simulink model "D_FB_J_classic_invdyn"  (R2020a)
settings: Solver=ode15s  StartTime=0.0  StopTime=T  MaxStep=0.01  RelTol=1e-3
values from neighbouring files (symbols this model uses):
  a1A = 0.5    [sim_D_FB_J.m]
  a1B = 0.5    [sim_D_FB_J.m]
  a2A = 0.5    [sim_D_FB_J.m]
  a2B = 0.5    [sim_D_FB_J.m]
  a3A = 0.5    [sim_D_FB_J.m]
  a3B = 0.5    [sim_D_FB_J.m]
  fv1A = 0    [sim_D_FB_J.m]
  fv1B = 0    [sim_D_FB_J.m]
  fv1p = 0    [sim_D_FB_J.m]
  fv2A = 0    [sim_D_FB_J.m]
  fv2B = 0    [sim_D_FB_J.m]
  fv2p = 0    [sim_D_FB_J.m]
  fv3A = 0    [sim_D_FB_J.m]
  fv3B = 0    [sim_D_FB_J.m]
  g0 = -9.81    [sim_D_FB_J.m]
  Ibzz = 12.1875    [sim_D_FB_J.m]
  Iczz = 33.7594    [sim_D_FB_J.m]
  Il1Azz = 0.108333    [sim_D_FB_J.m]
  Il1Bzz = 0.108333    [sim_D_FB_J.m]
  Il2Azz = 0.108333    [sim_D_FB_J.m]
  Il2Bzz = 0.108333    [sim_D_FB_J.m]
  Il3Azz = 0.108333    [sim_D_FB_J.m]
  Il3Bzz = 0.108333    [sim_D_FB_J.m]
  Kd = 5*eye(6)    [sim_D_FB_J.m]    (also in sim_second_arm_compensation.m; sim_second_arm_compensation2.m; sim_second_arm_compensation3.m = diag([5 5 5 1 1 1]))
  Kp = 5*eye(6)    [sim_D_FB_J.m]    (also in sim_second_arm_compensation.m; sim_second_arm_compensation2.m; sim_second_arm_compensation3.m = diag([5 5 5 1 1 1]))
  L = 3    [sim_D_FB_J.m]
  m_base = 100    [sim_D_FB_J.m]
  m_cavo = 45    [sim_D_FB_J.m]
  ml0 = 1000    [sim_D_FB_J.m]
  ml1A = 5    [sim_D_FB_J.m]
  ml1B = 5    [sim_D_FB_J.m]
  ml2A = 5    [sim_D_FB_J.m]
  ml2B = 5    [sim_D_FB_J.m]
  ml3A = 5    [sim_D_FB_J.m]
  ml3B = 5    [sim_D_FB_J.m]
  offA = -0.25    [sim_D_FB_J.m]
  offB = 0.25    [sim_D_FB_J.m]
  th1A_0 = -pi/2    (= -1.57079632679)    [sim_D_FB_J.m]    (also in sim_second_arm_compensation.m = 0; sim_second_arm_compensation2.m = 0; sim_second_arm_compensation3.m = -0.523598775598)
  th1B_0 = -pi/2    (= -1.57079632679)    [sim_D_FB_J.m]    (also in sim_second_arm_compensation.m = 0; sim_second_arm_compensation2.m = 0; sim_second_arm_compensation3.m = 0.523598775598)
  th2A_0 = -pi/8    (= -0.392699081699)    [sim_D_FB_J.m]    (also in sim_second_arm_compensation.m; sim_second_arm_compensation2.m; sim_second_arm_compensation3.m = 0.523598775598)
  th2B_0 = pi/8    (= 0.392699081699)    [sim_D_FB_J.m]    (also in sim_second_arm_compensation.m; sim_second_arm_compensation2.m; sim_second_arm_compensation3.m = -0.523598775598)
  th3A_0 = -pi/8    (= -0.392699081699)    [sim_D_FB_J.m]    (also in sim_second_arm_compensation.m; sim_second_arm_compensation2.m; sim_second_arm_compensation3.m = 0.523598775598)
  th3B_0 = pi/8    (= 0.392699081699)    [sim_D_FB_J.m]    (also in sim_second_arm_compensation.m; sim_second_arm_compensation2.m; sim_second_arm_compensation3.m = -0.523598775598)
undefined symbols (not defined in the file or in its folder): X, Y, Z
libraries: sm_lib x36, nesl_utility x25
(part 3 of 4)

== matlab function D_FB_J_classic_invdyn/Inverse dynamics ==
  data: y input; q input; qd input; tau output; m_cavo parameter; m_base parameter; ml1A parameter; ml2A parameter; ml3A parameter; ml1B parameter; ml2B parameter; ml3B parameter; L parameter; a1A parameter; a2A parameter; a3A parameter; a1B parameter; a2B parameter; a3B parameter; offA parameter; offB parameter; fv1p parameter; fv2p parameter; fv1A parameter; fv2A parameter; fv3A parameter; fv1B parameter; fv2B parameter; fv3B parameter; Ibzz parameter; Iczz parameter; Il1Azz parameter; Il1Bzz parameter; Il2Azz parameter; Il2Bzz parameter; Il3Azz parameter; Il3Bzz parameter; g0 parameter
function tau = fcn(y, q, qd, ...
                   m_cavo, m_base, ml1A, ml2A, ml3A, ml1B, ml2B, ml3B, ...
                   L, a1A, a2A, a3A, a1B, a2B, a3B, offA, offB, ...
                   fv1p, fv2p, fv1A, fv2A, fv3A, fv1B, fv2B, fv3B, ...
                   Ibzz, Iczz, Il1Azz, Il1Bzz, Il2Azz, Il2Bzz, Il3Azz, Il3Bzz, g0)

% Input
alfa = q(1);
beta = q(2);
th1A = q(3);
th2A = q(4);
th3A = q(5);
th1B = q(6);
th2B = q(7);
th3B = q(8);
dalfa = qd(1);
dbeta = qd(2);
dth1A = qd(3);
dth2A = qd(4);
dth3A = qd(5);
dth1B = qd(6);
dth2B = qd(7);
dth3B = qd(8);

% Matrice B
B = [ Ibzz + Iczz + Il1Azz + Il1Bzz + Il2Azz + Il2Bzz + Il3Azz + Il3Bzz + L^2*m_base + 0.2500*L^2*m_cavo + L^2*ml1A + L^2*ml1B + L^2*ml2A + L^2*ml2B + L^2*ml3A + L^2*ml3B + 0.2500*a1A^2*ml1A + a1A^2*ml2A + a1A^2*ml3A + 0.2500*a2A^2*ml2A + a2A^2*ml3A + 0.2500*a3A^2*ml3A + 0.2500*a1B^2*ml1B + a1B^2*ml2B + a1B^2*ml3B + 0.2500*a2B^2*ml2B + a2B^2*ml3B + 0.2500*a3B^2*ml3B + ml1A*offA^2 + ml2A*offA^2 + ml1B*offB^2 + ml3A*offA^2 + ml2B*offB^2 + ml3B*offB^2 + L*a1A*ml1A*cos(beta + th1A) + 2*L*a1A*ml2A*cos(beta + th1A) + 2*L*a1A*ml3A*cos(beta + th1A) + L*a1B*ml1B*cos(beta + th1B) + 2*L*a1B*ml2B*cos(beta + th1B) + 2*L*a1B*ml3B*cos(beta + th1B) + a1A*a3A*ml3A*cos(th2A + th3A) + a1B*a3B*ml3B*cos(th2B + th3B) + a2A*ml2A*offA*cos(th1A + th2A) + 2*a2A*ml3A*offA*cos(th1A + th2A) + a2B*ml2B*offB*cos(th1B + th2B) + 2*a2B*ml3B*offB*cos(th1B + th2B) + 2*L*ml1A*offA*cos(beta) + 2*L*ml2A*offA*cos(beta) + 2*L*ml1B*offB*cos(beta) + 2*L*ml3A*offA*cos(beta) + 2*L*ml2B*offB*cos(beta) + 2*L*ml3B*offB*cos(beta) + a1A*a2A*ml2A*cos(th2A) + 2*a1A*a2A*ml3A*cos(th2A) + a2A*a3A*ml3A*cos(th3A) + a1B*a2B*ml2B*cos(th2B) + 2*a1B*a2B*ml3B*cos(th2B) + a2B*a3B*ml3B*cos(th3B) + a1A*ml1A*offA*cos(th1A) + 2*a1A*ml2A*offA*cos(th1A) + 2*a1A*ml3A*offA*cos(th1A) + a1B*ml1B*offB*cos(th1B) + 2*a1B*ml2B*offB*cos(th1B) + 2*a1B*ml3B*offB*cos(th1B) + L*a2A*ml2A*cos(beta + th1A + th2A) + 2*L*a2A*ml3A*cos(beta + th1A + th2A) + L*a2B*ml2B*cos(beta + th1B + th2B) + 2*L*a2B*ml3B*cos(beta + th1B + th2B) + a3A*ml3A*offA*cos(th1A + th2A + th3A) + a3B*ml3B*offB*cos(th1B + th2B + th3B) + L*a3A*ml3A*cos(beta + th1A + th2A + th3A) + L*a3B*ml3B*cos(beta + th1B + th2B + th3B), Ibzz + Il1Azz + Il1Bzz + Il2Azz + Il2Bzz + Il3Azz + Il3Bzz + 0.2500*a1A^2*ml1A + a1A^2*ml2A + a1A^2*ml3A + 0.2500*a2A^2*ml2A + a2A^2*ml3A + 0.2500*a3A^2*ml3A + 0.2500*a1B^2*ml1B + a1B^2*ml2B + a1B^2*ml3B + 0.2500*a2B^2*ml2B + a2B^2*ml3B + 0.2500*a3B^2*ml3B + ml1A*offA^2 + ml2A*offA^2 + ml1B*offB^2 + ml3A*offA^2 + ml2B*offB^2 + ml3B*offB^2 + 0.5000*L*a1A*ml1A*cos(beta + th1A) + L*a1A*ml2A*cos(beta + th1A) + L*a1A*ml3A*cos(beta + th1A) + 0.5000*L*a1B*ml1B*cos(beta + th1B) + L*a1B*ml2B*cos(beta + th1B) + L*a1B*ml3B*cos(beta + th1B) + a1A*a3A*ml3A*cos(th2A + th3A) + a1B*a3B*ml3B*cos(th2B + th3B) + a2A*ml2A*offA*cos(th1A + th2A) + 2*a2A*ml3A*offA*cos(th1A + th2A) + a2B*ml2B*offB*cos(th1B + th2B) + 2*a2B*ml3B*offB*cos(th1B + th2B) + L*ml1A*offA*cos(beta) + L*ml2A*offA*cos(beta) + L*ml1B*offB*cos(beta) + L*ml3A*offA*cos(beta) + L*ml2B*offB*cos(beta) + L*ml3B*offB*cos(beta) + a1A*a2A*ml2A*cos(th2A) + 2*a1A*a2A*ml3A*cos(th2A) + a2A*a3A*ml3A*cos(th3A) + a1B*a2B*ml2B*cos(th2B) + 2*a1B*a2B*ml3B*cos(th2B) + a2B*a3B*ml3B*cos(th3B) + a1A*ml1A*offA*cos(th1A) + 2*a1A*ml2A*offA*cos(th1A) + 2*a1A*ml3A*offA*cos(th1A) + a1B*ml1B*offB*cos(th1B) + 2*a1B*ml2B*offB*cos(th1B) + 2*a1B*ml3B*offB*cos(th1B) + 0.5000*L*a2A*ml2A*cos(beta + th1A + th2A) + L*a2A*ml3A*cos(beta + th1A + th2A) + 0.5000*L*a2B*ml2B*cos(beta + th1B + th2B) + L*a2B*ml3B*cos(beta + th1B + th2B) + a3A*ml3A*offA*cos(th1A + th2A + th3A) + a3B*ml3B*offB*cos(th1B + th2B + th3B) + 0.5000*L*a3A*ml3A*cos(beta + th1A + th2A + th3A) + 0.5000*L*a3B*ml3B*cos(beta + th1B + th2B + th3B), Il1Azz + Il2Azz + Il3Azz + 0.2500*a1A^2*ml1A + a1A^2*ml2A + a1A^2*ml3A + 0.2500*a2A^2*ml2A + a2A^2*ml3A + 0.2500*a3A^2*ml3A + 0.5000*L*a1A*ml1A*cos(beta + th1A) + L*a1A*ml2A*cos(beta + th1A) + L*a1A*ml3A*cos(beta + th1A) + a1A*a3A*ml3A*cos(th2A + th3A) + 0.5000*a2A*ml2A*offA*cos(th1A + th2A) + a2A*ml3A*offA*cos(th1A + th2A) + a1A*a2A*ml2A*cos(th2A) + 2*a1A*a2A*ml3A*cos(th2A) + a2A*a3A*ml3A*cos(th3A) + 0.5000*a1A*ml1A*offA*cos(th1A) + a1A*ml2A*offA*cos(th1A) + a1A*ml3A*offA*cos(th1A) + 0.5000*L*a2A*ml2A*cos(beta + th1A + th2A) + L*a2A*ml3A*cos(beta + th1A + th2A) + 0.5000*a3A*ml3A*offA*cos(th1A + th2A + th3A) + 0.5000*L*a3A*ml3A*cos(beta + th1A + th2A + th3A), Il2Azz + Il3Azz + 0.2500*a2A^2*ml2A + a2A^2*ml3A + 0.2500*a3A^2*ml3A + 0.5000*a1A*a3A*ml3A*cos(th2A + th3A) + 0.5000*a2A*ml2A*offA*cos(th1A + th2A) + a2A*ml3A*offA*cos(th1A + th2A) + 0.5000*a1A*a2A*ml2A*cos(th2A) + a1A*a2A*ml3A*cos(th2A) + a2A*a3A*ml3A*cos(th3A) + 0.5000*L*a2A*ml2A*cos(beta + th1A + th2A) + L*a2A*ml3A*cos(beta + th1A + th2A) + 0.5000*a3A*ml3A*offA*cos(th1A + th2A + th3A) + 0.5000*L*a3A*ml3A*cos(beta + th1A + th2A + th3A), Il3Azz + 0.2500*a3A^2*ml3A + 0.5000*a1A*a3A*ml3A*cos(th2A + th3A) + 0.5000*a2A*a3A*ml3A*cos(th3A) + 0.5000*a3A*ml3A*offA*cos(th1A + th2A + th3A) + 0.5000*L*a3A*ml3A*cos(beta + th1A + th2A + th3A), Il1Bzz + Il2Bzz + Il3Bzz + 0.2500*a1B^2*ml1B + a1B^2*ml2B + a1B^2*ml3B + 0.2500*a2B^2*ml2B + a2B^2*ml3B + 0.2500*a3B^2*ml3B + 0.5000*L*a1B*ml1B*cos(beta + th1B) + L*a1B*ml2B*cos(beta + th1B) + L*a1B*ml3B*cos(beta + th1B) + a1B*a3B*ml3B*cos(th2B + th3B) + 0.5000*a2B*ml2B*offB*cos(th1B + th2B) + a2B*ml3B*offB*cos(th1B + th2B) + a1B*a2B*ml2B*cos(th2B) + 2*a1B*a2B*ml3B*cos(th2B) + a2B*a3B*ml3B*cos(th3B) + 0.5000*a1B*ml1B*offB*cos(th1B) + a1B*ml2B*offB*cos(th1B) + a1B*ml3B*offB*cos(th1B) + 0.5000*L*a2B*ml2B*cos(beta + th1B + th2B) + L*a2B*ml3B*cos(beta + th1B + th2B) + 0.5000*a3B*ml3B*offB*cos(th1B + th2B + th3B) + 0.5000*L*a3B*ml3B*cos(beta + th1B + th2B + th3B), Il2Bzz + Il3Bzz + 0.2500*a2B^2*ml2B + a2B^2*ml3B + 0.2500*a3B^2*ml3B + 0.5000*a1B*a3B*ml3B*cos(th2B + th3B) + 0.5000*a2B*ml2B*offB*cos(th1B + th2B) + a2B*ml3B*offB*cos(th1B + th2B) + 0.5000*a1B*a2B*ml2B*cos(th2B) + a1B*a2B*ml3B*cos(th2B) + a2B*a3B*ml3B*cos(th3B) + 0.5000*L*a2B*ml2B*cos(beta + th1B + th2B) + L*a2B*ml3B*cos(beta + th1B + th2B) + 0.5000*a3B*ml3B*offB*cos(th1B + th2B + th3B) + 0.5000*L*a3B*ml3B*cos(beta + th1B + th2B + th3B), Il3Bzz + 0.2500*a3B^2*ml3B + 0.5000*a1B*a3B*ml3B*cos(th2B + th3B) + 0.5000*a2B*a3B*ml3B*cos(th3B) + 0.5000*a3B*ml3B*offB*cos(th1B + th2B + th3B) + 0.5000*L*a3B*ml3B*cos(beta + th1B + th2B + th3B); ...
                                                                                              Ibzz + Il1Azz + Il1Bzz + Il2Azz + Il2Bzz + Il3Azz + Il3Bzz + 0.2500*a1A^2*ml1A + a1A^2*ml2A + a1A^2*ml3A + 0.2500*a2A^2*ml2A + a2A^2*ml3A + 0.2500*a3A^2*ml3A + 0.2500*a1B^2*ml1B + a1B^2*ml2B + a1B^2*ml3B + 0.2500*a2B^2*ml2B + a2B^2*ml3B + 0.2500*a3B^2*ml3B + ml1A*offA^2 + ml2A*offA^2 + ml1B*offB^2 + ml3A*offA^2 + ml2B*offB^2 + ml3B*offB^2 + 0.5000*L*a1A*ml1A*cos(beta + th1A) + L*a1A*ml2A*cos(beta + th1A) + L*a1A*ml3A*cos(beta + th1A) + 0.5000*L*a1B*ml1B*cos(beta + th1B) + L*a1B*ml2B*cos(beta + th1B) + L*a1B*ml3B*cos(beta + th1B) + a1A*a3A*ml3A*cos(th2A + th3A) + a1B*a3B*ml3B*cos(th2B + th3B) + a2A*ml2A*offA*cos(th1A + th2A) + 2*a2A*ml3A*offA*cos(th1A + th2A) + a2B*ml2B*offB*cos(th1B + th2B) + 2*a2B*ml3B*offB*cos(th1B + th2B) + L*ml1A*offA*cos(beta) + L*ml2A*offA*cos(beta) + L*ml1B*offB*cos(beta) + L*ml3A*offA*cos(beta) + L*ml2B*offB*cos(beta) + L*ml3B*offB*cos(beta) + a1A*a2A*ml2A*cos(th2A) + 2*a1A*a2A*ml3A*cos(th2A) + a2A*a3A*ml3A*cos(th3A) + a1B*a2B*ml2B*cos(th2B) + 2*a1B*a2B*ml3B*cos(th2B) + a2B*a3B*ml3B*cos(th3B) + a1A*ml1A*offA*cos(th1A) + 2*a1A*ml2A*offA*cos(th1A) + 2*a1A*ml3A*offA*cos(th1A) + a1B*ml1B*offB*cos(th1B) + 2*a1B*ml2B*offB*cos(th1B) + 2*a1B*ml3B*offB*cos(th1B) + 0.5000*L*a2A*ml2A*cos(beta + th1A + th2A) + L*a2A*ml3A*cos(beta + th1A + th2A) + 0.5000*L*a2B*ml2B*cos(beta + th1B + th2B) + L*a2B*ml3B*cos(beta + th1B + th2B) + a3A*ml3A*offA*cos(th1A + th2A + th3A) + a3B*ml3B*offB*cos(th1B + th2B + th3B) + 0.5000*L*a3A*ml3A*cos(beta + th1A + th2A + th3A) + 0.5000*L*a3B*ml3B*cos(beta + th1B + th2B + th3B),                                                                                                                                                                                                                                                                                                                                                                                                                                                                                                                                                                                                                           Ibzz + Il1Azz + Il1Bzz + Il2Azz + Il2Bzz + Il3Azz + Il3Bzz + 0.2500*a1A^2*ml1A + a1A^2*ml2A + a1A^2*ml3A + 0.2500*a2A^2*ml2A + a2A^2*ml3A + 0.2500*a3A^2*ml3A + 0.2500*a1B^2*ml1B + a1B^2*ml2B + a1B^2*ml3B + 0.2500*a2B^2*ml2B + a2B^2*ml3B + 0.2500*a3B^2*ml3B + ml1A*offA^2 + ml2A*offA^2 + ml1B*offB^2 + ml3A*offA^2 + ml2B*offB^2 + ml3B*offB^2 + a1A*a3A*ml3A*cos(th2A + th3A) + a1B*a3B*ml3B*cos(th2B + th3B) + a2A*ml2A*offA*cos(th1A + th2A) + 2*a2A*ml3A*offA*cos(th1A + th2A) + a2B*ml2B*offB*cos(th1B + th2B) + 2*a2B*ml3B*offB*cos(th1B + th2B) + a1A*a2A*ml2A*cos(th2A) + 2*a1A*a2A*ml3A*cos(th2A) + a2A*a3A*ml3A*cos(th3A) + a1B*a2B*ml2B*cos(th2B) + 2*a1B*a2B*ml3B*cos(th2B) + a2B*a3B*ml3B*cos(th3B) + a1A*ml1A*offA*cos(th1A) + 2*a1A*ml2A*offA*cos(th1A) + 2*a1A*ml3A*offA*cos(th1A) + a1B*ml1B*offB*cos(th1B) + 2*a1B*ml2B*offB*cos(th1B) + 2*a1B*ml3B*offB*cos(th1B) + a3A*ml3A*offA*cos(th1A + th2A + th3A) + a3B*ml3B*offB*cos(th1B + th2B + th3B),                                                                                                                                                                                                                                      Il1Azz + Il2Azz + Il3Azz + 0.2500*a1A^2*ml1A + a1A^2*ml2A + a1A^2*ml3A + 0.2500*a2A^2*ml2A + a2A^2*ml3A + 0.2500*a3A^2*ml3A + a1A*a3A*ml3A*cos(th2A + th3A) + 0.5000*a2A*ml2A*offA*cos(th1A + th2A) + a2A*ml3A*offA*cos(th1A + th2A) + a1A*a2A*ml2A*cos(th2A) + 2*a1A*a2A*ml3A*cos(th2A) + a2A*a3A*ml3A*cos(th3A) + 0.5000*a1A*ml1A*offA*cos(th1A) + a1A*ml2A*offA*cos(th1A) + a1A*ml3A*offA*cos(th1A) + 0.5000*a3A*ml3A*offA*cos(th1A + th2A + th3A),                                                                                                                                     Il2Azz + Il3Azz + 0.2500*a2A^2*ml2A + a2A^2*ml3A + 0.2500*a3A^2*ml3A + 0.5000*a1A*a3A*ml3A*cos(th2A + th3A) + 0.5000*a2A*ml2A*offA*cos(th1A + th2A) + a2A*ml3A*offA*cos(th1A + th2A) + 0.5000*a1A*a2A*ml2A*cos(th2A) + a1A*a2A*ml3A*cos(th2A) + a2A*a3A*ml3A*cos(th3A) + 0.5000*a3A*ml3A*offA*cos(th1A + th2A + th3A),                                                    Il3Azz + 0.2500*a3A^2*ml3A + 0.5000*a1A*a3A*ml3A*cos(th2A + th3A) + 0.5000*a2A*a3A*ml3A*cos(th3A) + 0.5000*a3A*ml3A*offA*cos(th1A + th2A + th3A),                                                                                                                                                                                                                                      Il1Bzz + Il2Bzz + Il3Bzz + 0.2500*a1B^2*ml1B + a1B^2*ml2B + a1B^2*ml3B + 0.2500*a2B^2*ml2B + a2B^2*ml3B + 0.2500*a3B^2*ml3B + a1B*a3B*ml3B*cos(th2B + th3B) + 0.5000*a2B*ml2B*offB*cos(th1B + th2B) + a2B*ml3B*offB*cos(th1B + th2B) + a1B*a2B*ml2B*cos(th2B) + 2*a1B*a2B*ml3B*cos(th2B) + a2B*a3B*ml3B*cos(th3B) + 0.5000*a1B*ml1B*offB*cos(th1B) + a1B*ml2B*offB*cos(th1B) + a1B*ml3B*offB*cos(th1B) + 0.5000*a3B*ml3B*offB*cos(th1B + th2B + th3B),                                                                                                                                     Il2Bzz + Il3Bzz + 0.2500*a2B^2*ml2B + a2B^2*ml3B + 0.2500*a3B^2*ml3B + 0.5000*a1B*a3B*ml3B*cos(th2B + th3B) + 0.5000*a2B*ml2B*offB*cos(th1B + th2B) + a2B*ml3B*offB*cos(th1B + th2B) + 0.5000*a1B*a2B*ml2B*cos(th2B) + a1B*a2B*ml3B*cos(th2B) + a2B*a3B*ml3B*cos(th3B) + 0.5000*a3B*ml3B*offB*cos(th1B + th2B + th3B),                                                    Il3Bzz + 0.2500*a3B^2*ml3B + 0.5000*a1B*a3B*ml3B*cos(th2B + th3B) + 0.5000*a2B*a3B*ml3B*cos(th3B) + 0.5000*a3B*ml3B*offB*cos(th1B + th2B + th3B); ...
                                                                                                                                                                                                                                                                                                                                                                                                                                                                                                                                                                                                                                                                                                                                                                                                                                                                                                                                                                                                        Il1Azz + Il2Azz + Il3Azz + 0.2500*a1A^2*ml1A + a1A^2*ml2A + a1A^2*ml3A + 0.2500*a2A^2*ml2A + a2A^2*ml3A + 0.2500*a3A^2*ml3A + 0.5000*L*a1A*ml1A*cos(beta + th1A) + L*a1A*ml2A*cos(beta + th1A) + L*a1A*ml3A*cos(beta + th1A) + a1A*a3A*ml3A*cos(th2A + th3A) + 0.5000*a2A*ml2A*offA*cos(th1A + th2A) + a2A*ml3A*offA*cos(th1A + th2A) + a1A*a2A*ml2A*cos(th2A) + 2*a1A*a2A*ml3A*cos(th2A) + a2A*a3A*ml3A*cos(th3A) + 0.5000*a1A*ml1A*offA*cos(th1A) + a1A*ml2A*offA*cos(th1A) + a1A*ml3A*offA*cos(th1A) + 0.5000*L*a2A*ml2A*cos(beta + th1A + th2A) + L*a2A*ml3A*cos(beta + th1A + th2A) + 0.5000*a3A*ml3A*offA*cos(th1A + th2A + th3A) + 0.5000*L*a3A*ml3A*cos(beta + th1A + th2A + th3A),                                                                                                                                                                                                                                                                                                                                                                                                                                                                                                                                                                                                                                                                                                                                                                                                                                                                                                                                                                                                                                                                                                                                                Il1Azz + Il2Azz + Il3Azz + 0.2500*a1A^2*ml1A + a1A^2*ml2A + a1A^2*ml3A + 0.2500*a2A^2*ml2A + a2A^2*ml3A + 0.2500*a3A^2*ml3A + a1A*a3A*ml3A*cos(th2A + th3A) + 0.5000*a2A*ml2A*offA*cos(th1A + th2A) + a2A*ml3A*offA*cos(th1A + th2A) + a1A*a2A*ml2A*cos(th2A) + 2*a1A*a2A*ml3A*cos(th2A) + a2A*a3A*ml3A*cos(th3A) + 0.5000*a1A*ml1A*offA*cos(th1A) + a1A*ml2A*offA*cos(th1A) + a1A*ml3A*offA*cos(th1A) + 0.5000*a3A*ml3A*offA*cos(th1A + th2A + th3A),                                                                                                                                                                                                                                                                                                                                                                                                                                                   Il1Azz + Il2Azz + Il3Azz + 0.2500*a1A^2*ml1A + a1A^2*ml2A + a1A^2*ml3A + 0.2500*a2A^2*ml2A + a2A^2*ml3A + 0.2500*a3A^2*ml3A + a1A*a3A*ml3A*cos(th2A + th3A) + a1A*a2A*ml2A*cos(th2A) + 2*a1A*a2A*ml3A*cos(th2A) + a2A*a3A*ml3A*cos(th3A),                                                                                                                                                                                                                                                             Il2Azz + Il3Azz + 0.2500*a2A^2*ml2A + a2A^2*ml3A + 0.2500*a3A^2*ml3A + 0.5000*a1A*a3A*ml3A*cos(th2A + th3A) + 0.5000*a1A*a2A*ml2A*cos(th2A) + a1A*a2A*ml3A*cos(th2A) + a2A*a3A*ml3A*cos(th3A),                                                                                                   Il3Azz + 0.2500*a3A^2*ml3A + 0.5000*a1A*a3A*ml3A*cos(th2A + th3A) + 0.5000*a2A*a3A*ml3A*cos(th3A),                                                                                                                                                                                                                                                                                                                                                                                                                                                                                                                                                                                                                                                                                          0,                                                                                                                                                                                                                                                                                                                                                                                                                                                         0,                                                                                                                                                                                                   0; ...
                                                                                                                                                                                                                                                                                                                                                                                                                                                                                                                                                                                                                                                                                                                                                                                                                                                                                                                                                                                                                                                                                                                                                                                                                                         Il2Azz + Il3Azz + 0.2500*a2A^2*ml2A + a2A^2*ml3A + 0.2500*a3A^2*ml3A + 0.5000*a1A*a3A*ml3A*cos(th2A + th3A) + 0.5000*a2A*ml2A*offA*cos(th1A + th2A) + a2A*ml3A*offA*cos(th1A + th2A) + 0.5000*a1A*a2A*ml2A*cos(th2A) + a1A*a2A*ml3A*cos(th2A) + a2A*a3A*ml3A*cos(th3A) + 0.5000*L*a2A*ml2A*cos(beta + th1A + th2A) + L*a2A*ml3A*cos(beta + th1A + th2A) + 0.5000*a3A*ml3A*offA*cos(th1A + th2A + th3A) + 0.5000*L*a3A*ml3A*cos(beta + th1A + th2A + th3A),                                                                                                                                                                                                                                                                                                                                                                                                                                                                                                                                                                                                                                                                                                                                                                                                                                                                                                                                                                                                                                                                                                                                                                                                                                                                                Il2Azz + Il3Azz + 0.2500*a2A^2*ml2A + a2A^2*ml3A + 0.2500*a3A^2*ml3A + 0.5000*a1A*a3A*ml3A*cos(th2A + th3A) + 0.5000*a2A*ml2A*offA*cos(th1A + th2A) + a2A*ml3A*offA*cos(th1A + th2A) + 0.5000*a1A*a2A*ml2A*cos(th2A) + a1A*a2A*ml3A*cos(th2A) + a2A*a3A*ml3A*cos(th3A) + 0.5000*a3A*ml3A*offA*cos(th1A + th2A + th3A),                                                                                                                                                                                                                                                                                                                                                                                                                                                                                              Il2Azz + Il3Azz + 0.2500*a2A^2*ml2A + a2A^2*ml3A + 0.2500*a3A^2*ml3A + 0.5000*a1A*a3A*ml3A*cos(th2A + th3A) + 0.5000*a1A*a2A*ml2A*cos(th2A) + a1A*a2A*ml3A*cos(th2A) + a2A*a3A*ml3A*cos(th3A),                                                                                                                                                                                                                                                                                                                                                             Il2Azz + Il3Azz + 0.2500*a2A^2*ml2A + a2A^2*ml3A + 0.2500*a3A^2*ml3A + a2A*a3A*ml3A*cos(th3A),                                                                                                                                          0.2500*ml3A*a3A^2 + 0.5000*a2A*ml3A*cos(th3A)*a3A + Il3Azz,                                                                                                                                                                                                                                                                                                                                                                                                                                                                                                                                                                                                                                                                                          0,                                                                                                                                                                                                                                                                                                                                                                                                                                                         0,                                                                                                                                                                                                   0; ...
                                                                                                                                                                                                                                                                                                                                                                                                                                                                                                                                                                                                                                                                                                                                                                                                                                                                                                                                                                                                                                                                                                                                                                                                                                                                                                                                                                                                                                                                                               Il3Azz + 0.2500*a3A^2*ml3A + 0.5000*a1A*a3A*ml3A*cos(th2A + th3A) + 0.5000*a2A*a3A*ml3A*cos(th3A) + 0.5000*a3A*ml3A*offA*cos(th1A + th2A + th3A) + 0.5000*L*a3A*ml3A*cos(beta + th1A + th2A + th3A),                                                                                                                                                                                                                                                                                                                                                                                                                                                                                                                                                                                                                                                                                                                                                                                                                                                                                                                                                                                                                                                                                                                                                                                                                                                                                                                                                                                                                                                     Il3Azz + 0.2500*a3A^2*ml3A + 0.5000*a1A*a3A*ml3A*cos(th2A + th3A) + 0.5000*a2A*a3A*ml3A*cos(th3A) + 0.5000*a3A*ml3A*offA*cos(th1A + th2A + th3A),                                                                                                                                                                                                                                                                                                                                                                                                                                                                                                                                                                                          Il3Azz + 0.2500*a3A^2*ml3A + 0.5000*a1A*a3A*ml3A*cos(th2A + th3A) + 0.5000*a2A*a3A*ml3A*cos(th3A),                                                                                                                                                                                                                                                                                                                                                                                                0.2500*ml3A*a3A^2 + 0.5000*a2A*ml3A*cos(th3A)*a3A + Il3Azz,                                                                                                                                                                          0.2500*ml3A*a3A^2 + Il3Azz,                                                                                                                                                                                                                                                                                                                                                                                                                                                                                                                                                                                                                                                                                          0,                                                                                                                                                                                                                                                                                                                                                                                                                                                         0,                                                                                                                                                                                                   0; ...
                                                                                                                                                                                                                                                                                                                                                                                                                                                                                                                                                                                                                                                                                                                                                                                                                                                                                                                                                                                                        Il1Bzz + Il2Bzz + Il3Bzz + 0.2500*a1B^2*ml1B + a1B^2*ml2B + a1B^2*ml3B + 0.2500*a2B^2*ml2B + a2B^2*ml3B + 0.2500*a3B^2*ml3B + 0.5000*L*a1B*ml1B*cos(beta + th1B) + L*a1B*ml2B*cos(beta + th1B) + L*a1B*ml3B*cos(beta + th1B) + a1B*a3B*ml3B*cos(th2B + th3B) + 0.5000*a2B*ml2B*offB*cos(th1B + th2B) + a2B*ml3B*offB*cos(th1B + th2B) + a1B*a2B*ml2B*cos(th2B) + 2*a1B*a2B*ml3B*cos(th2B) + a2B*a3B*ml3B*cos(th3B) + 0.5000*a1B*ml1B*offB*cos(th1B) + a1B*ml2B*offB*cos(th1B) + a1B*ml3B*offB*cos(th1B) + 0.5000*L*a2B*ml2B*cos(beta + th1B + th2B) + L*a2B*ml3B*cos(beta + th1B + th2B) + 0.5000*a3B*ml3B*offB*cos(th1B + th2B + th3B) + 0.5000*L*a3B*ml3B*cos(beta + th1B + th2B + th3B),                                                                                                                                                                                                                                                                                                                                                                                                                                                                                                                                                                                                                                                                                                                                                                                                                                                                                                                                                                                                                                                                                                                                                Il1Bzz + Il2Bzz + Il3Bzz + 0.2500*a1B^2*ml1B + a1B^2*ml2B + a1B^2*ml3B + 0.2500*a2B^2*ml2B + a2B^2*ml3B + 0.2500*a3B^2*ml3B + a1B*a3B*ml3B*cos(th2B + th3B) + 0.5000*a2B*ml2B*offB*cos(th1B + th2B) + a2B*ml3B*offB*cos(th1B + th2B) + a1B*a2B*ml2B*cos(th2B) + 2*a1B*a2B*ml3B*cos(th2B) + a2B*a3B*ml3B*cos(th3B) + 0.5000*a1B*ml1B*offB*cos(th1B) + a1B*ml2B*offB*cos(th1B) + a1B*ml3B*offB*cos(th1B) + 0.5000*a3B*ml3B*offB*cos(th1B + th2B + th3B),                                                                                                                                                                                                                                                                                                                                                                                                                                                                                                                                                                                                                                                                                          0,                                                                                                                                                                                                                                                                                                                                                                                                                                                         0,                                                                                                                                                                                                   0,                                                                                                                                                                                                                                                                                                                                                                                                                                                   Il1Bzz + Il2Bzz + Il3Bzz + 0.2500*a1B^2*ml1B + a1B^2*ml2B + a1B^2*ml3B + 0.2500*a2B^2*ml2B + a2B^2*ml3B + 0.2500*a3B^2*ml3B + a1B*a3B*ml3B*cos(th2B + th3B) + a1B*a2B*ml2B*cos(th2B) + 2*a1B*a2B*ml3B*cos(th2B) + a2B*a3B*ml3B*cos(th3B),                                                                                                                                                                                                                                                             Il2Bzz + Il3Bzz + 0.2500*a2B^2*ml2B + a2B^2*ml3B + 0.2500*a3B^2*ml3B + 0.5000*a1B*a3B*ml3B*cos(th2B + th3B) + 0.5000*a1B*a2B*ml2B*cos(th2B) + a1B*a2B*ml3B*cos(th2B) + a2B*a3B*ml3B*cos(th3B),                                                                                                   Il3Bzz + 0.2500*a3B^2*ml3B + 0.5000*a1B*a3B*ml3B*cos(th2B + th3B) + 0.5000*a2B*a3B*ml3B*cos(th3B); ...
                                                                                                                                                                                                                                                                                                                                                                                                                                                                                                                                                                                                                                                                                                                                                                                                                                                                                                                                                                                                                                                                                                                                                                                                                                         Il2Bzz + Il3Bzz + 0.2500*a2B^2*ml2B + a2B^2*ml3B + 0.2500*a3B^2*ml3B + 0.5000*a1B*a3B*ml3B*cos(th2B + th3B) + 0.5000*a2B*ml2B*offB*cos(th1B + th2B) + a2B*ml3B*offB*cos(th1B + th2B) + 0.5000*a1B*a2B*ml2B*cos(th2B) + a1B*a2B*ml3B*cos(th2B) + a2B*a3B*ml3B*cos(th3B) + 0.5000*L*a2B*ml2B*cos(beta + th1B + th2B) + L*a2B*ml3B*cos(beta + th1B + th2B) + 0.5000*a3B*ml3B*offB*cos(th1B + th2B + th3B) + 0.5000*L*a3B*ml3B*cos(beta + th1B + th2B + th3B),                                                                                                                                                                                                                                                                                                                                                                                                                                                                                                                                                                                                                                                                                                                                                                                                                                                                                                                                                                                                                                                                                                                                                                                                                                                                                Il2Bzz + Il3Bzz + 0.2500*a2B^2*ml2B + a2B^2*ml3B + 0.2500*a3B^2*ml3B + 0.5000*a1B*a3B*ml3B*cos(th2B + th3B) + 0.5000*a2B*ml2B*offB*cos(th1B + th2B) + a2B*ml3B*offB*cos(th1B + th2B) + 0.5000*a1B*a2B*ml2B*cos(th2B) + a1B*a2B*ml3B*cos(th2B) + a2B*a3B*ml3B*cos(th3B) + 0.5000*a3B*ml3B*offB*cos(th1B + th2B + th3B),                                                                                                                                                                                                                                                                                                                                                                                                                                                                                                                                                                                                                                                                                          0,                                                                                                                                                                                                                                                                                                                                                                                                                                                         0,                                                                                                                                                                                                   0,                                                                                                                                                                                                                                                                                                                                                                                                                                                                                              Il2Bzz + Il3Bzz + 0.2500*a2B^2*ml2B + a2B^2*ml3B + 0.2500*a3B^2*ml3B + 0.5000*a1B*a3B*ml3B*cos(th2B + th3B) + 0.5000*a1B*a2B*ml2B*cos(th2B) + a1B*a2B*ml3B*cos(th2B) + a2B*a3B*ml3B*cos(th3B),                                                                                                                                                                                                                                                                                                                                                             Il2Bzz + Il3Bzz + 0.2500*a2B^2*ml2B + a2B^2*ml3B + 0.2500*a3B^2*ml3B + a2B*a3B*ml3B*cos(th3B),                                                                                                                                          0.2500*ml3B*a3B^2 + 0.5000*a2B*ml3B*cos(th3B)*a3B + Il3Bzz; ...
                                                                                                                                                                                                                                                                                                                                                                                                                                                                                                                                                                                                                                                                                                                                                                                                                                                                                                                                                                                                                                                                                                                                                                                                                                                                                                                                                                                                                                                                                               Il3Bzz + 0.2500*a3B^2*ml3B + 0.5000*a1B*a3B*ml3B*cos(th2B + th3B) + 0.5000*a2B*a3B*ml3B*cos(th3B) + 0.5000*a3B*ml3B*offB*cos(th1B + th2B + th3B) + 0.5000*L*a3B*ml3B*cos(beta + th1B + th2B + th3B),                                                                                                                                                                                                                                                                                                                                                                                                                                                                                                                                                                                                                                                                                                                                                                                                                                                                                                                                                                                                                                                                                                                                                                                                                                                                                                                                                                                                                                                     Il3Bzz + 0.2500*a3B^2*ml3B + 0.5000*a1B*a3B*ml3B*cos(th2B + th3B) + 0.5000*a2B*a3B*ml3B*cos(th3B) + 0.5000*a3B*ml3B*offB*cos(th1B + th2B + th3B),                                                                                                                                                                                                                                                                                                                                                                                                                                                                                                                                                                                                                                                                                          0,                                                                                                                                                                                                                                                                                                                                                                                                                                                         0,                                                                                                                                                                                                   0,                                                                                                                                                                                                                                                                                                                                                                                                                                                                                                                                                                                          Il3Bzz + 0.2500*a3B^2*ml3B + 0.5000*a1B*a3B*ml3B*cos(th2B + th3B) + 0.5000*a2B*a3B*ml3B*cos(th3B),                                                                                                                                                                                                                                                                                                                                                                                                0.2500*ml3B*a3B^2 + 0.5000*a2B*ml3B*cos(th3B)*a3B + Il3Bzz,                                                                                                                                                                          0.2500*ml3B*a3B^2 + Il3Bzz];
 
% Matrice C
C = [ - 0.5000*a3A*dth1A*ml3A*offA*sin(th1A + th2A + th3A) - 0.5000*a3A*dth2A*ml3A*offA*sin(th1A + th2A + th3A) - 0.5000*a3A*dth3A*ml3A*offA*sin(th1A + th2A + th3A) - 0.5000*a3B*dth1B*ml3B*offB*sin(th1B + th2B + th3B) - 0.5000*a3B*dth2B*ml3B*offB*sin(th1B + th2B + th3B) - 0.5000*a3B*dth3B*ml3B*offB*sin(th1B + th2B + th3B) - 0.5000*L*a3A*dbeta*ml3A*sin(beta + th1A + th2A + th3A) - 0.5000*L*a3B*dbeta*ml3B*sin(beta + th1B + th2B + th3B) - 0.5000*L*a3A*dth1A*ml3A*sin(beta + th1A + th2A + th3A) - 0.5000*L*a3A*dth2A*ml3A*sin(beta + th1A + th2A + th3A) - 0.5000*L*a3A*dth3A*ml3A*sin(beta + th1A + th2A + th3A) - 0.5000*L*a3B*dth1B*ml3B*sin(beta + th1B + th2B + th3B) - 0.5000*L*a3B*dth2B*ml3B*sin(beta + th1B + th2B + th3B) - 0.5000*L*a3B*dth3B*ml3B*sin(beta + th1B + th2B + th3B) - 0.5000*L*a1A*dbeta*ml1A*sin(beta + th1A) - L*a1A*dbeta*ml2A*sin(beta + th1A) - L*a1A*dbeta*ml3A*sin(beta + th1A) - 0.5000*L*a1B*dbeta*ml1B*sin(beta + th1B) - L*a1B*dbeta*ml2B*sin(beta + th1B) - L*a1B*dbeta*ml3B*sin(beta + th1B) - 0.5000*L*a1A*dth1A*ml1A*sin(beta + th1A) - L*a1A*dth1A*ml2A*sin(beta + th1A) - L*a1A*dth1A*ml3A*sin(beta + th1A) - 0.5000*L*a1B*dth1B*ml1B*sin(beta + th1B) - L*a1B*dth1B*ml2B*sin(beta + th1B) - L*a1B*dth1B*ml3B*sin(beta + th1B) - 0.5000*a1A*a3A*dth2A*ml3A*sin(th2A + th3A) - 0.5000*a1A*a3A*dth3A*ml3A*sin(th2A + th3A) - 0.5000*a1B*a3B*dth2B*ml3B*sin(th2B + th3B) - 0.5000*a1B*a3B*dth3B*ml3B*sin(th2B + th3B) - 0.5000*a2A*dth1A*ml2A*offA*sin(th1A + th2A) - a2A*dth1A*ml3A*offA*sin(th1A + th2A) - 0.5000*a2A*dth2A*ml2A*offA*sin(th1A + th2A) - a2A*dth2A*ml3A*offA*sin(th1A + th2A) - 0.5000*a2B*dth1B*ml2B*offB*sin(th1B + th2B) - a2B*dth1B*ml3B*offB*sin(th1B + th2B) - 0.5000*a2B*dth2B*ml2B*offB*sin(th1B + th2B) - a2B*dth2B*ml3B*offB*sin(th1B + th2B) - L*dbeta*ml1A*offA*sin(beta) - L*dbeta*ml2A*offA*sin(beta) - L*dbeta*ml1B*offB*sin(beta) - L*dbeta*ml3A*offA*sin(beta) - L*dbeta*ml2B*offB*sin(beta) - L*dbeta*ml3B*offB*sin(beta) - 0.5000*a1A*a2A*dth2A*ml2A*sin(th2A) - a1A*a2A*dth2A*ml3A*sin(th2A) - 0.5000*a2A*a3A*dth3A*ml3A*sin(th3A) - 0.5000*a1B*a2B*dth2B*ml2B*sin(th2B) - a1B*a2B*dth2B*ml3B*sin(th2B) - 0.5000*a2B*a3B*dth3B*ml3B*sin(th3B) - 0.5000*a1A*dth1A*ml1A*offA*sin(th1A) - a1A*dth1A*ml2A*offA*sin(th1A) - a1A*dth1A*ml3A*offA*sin(th1A) - 0.5000*a1B*dth1B*ml1B*offB*sin(th1B) - a1B*dth1B*ml2B*offB*sin(th1B) - a1B*dth1B*ml3B*offB*sin(th1B) - 0.5000*L*a2A*dbeta*ml2A*sin(beta + th1A + th2A) - L*a2A*dbeta*ml3A*sin(beta + th1A + th2A) - 0.5000*L*a2B*dbeta*ml2B*sin(beta + th1B + th2B) - L*a2B*dbeta*ml3B*sin(beta + th1B + th2B) - 0.5000*L*a2A*dth1A*ml2A*sin(beta + th1A + th2A) - L*a2A*dth1A*ml3A*sin(beta + th1A + th2A) - 0.5000*L*a2A*dth2A*ml2A*sin(beta + th1A + th2A) - L*a2A*dth2A*ml3A*sin(beta + th1A + th2A) - 0.5000*L*a2B*dth1B*ml2B*sin(beta + th1B + th2B) - L*a2B*dth1B*ml3B*sin(beta + th1B + th2B) - 0.5000*L*a2B*dth2B*ml2B*sin(beta + th1B + th2B) - L*a2B*dth2B*ml3B*sin(beta + th1B + th2B), - 0.5000*a3A*dth1A*ml3A*offA*sin(th1A + th2A + th3A) - 0.5000*a3A*dth2A*ml3A*offA*sin(th1A + th2A + th3A) - 0.5000*a3A*dth3A*ml3A*offA*sin(th1A + th2A + th3A) - 0.5000*a3B*dth1B*ml3B*offB*sin(th1B + th2B + th3B) - 0.5000*a3B*dth2B*ml3B*offB*sin(th1B + th2B + th3B) - 0.5000*a3B*dth3B*ml3B*offB*sin(th1B + th2B + th3B) - 0.5000*L*a3A*dalfa*ml3A*sin(beta + th1A + th2A + th3A) - 0.5000*L*a3B*dalfa*ml3B*sin(beta + th1B + th2B + th3B) - 0.5000*L*a3A*dbeta*ml3A*sin(beta + th1A + th2A + th3A) - 0.5000*L*a3B*dbeta*ml3B*sin(beta + th1B + th2B + th3B) - 0.5000*L*a3A*dth1A*ml3A*sin(beta + th1A + th2A + th3A) - 0.5000*L*a3A*dth2A*ml3A*sin(beta + th1A + th2A + th3A) - 0.5000*L*a3A*dth3A*ml3A*sin(beta + th1A + th2A + th3A) - 0.5000*L*a3B*dth1B*ml3B*sin(beta + th1B + th2B + th3B) - 0.5000*L*a3B*dth2B*ml3B*sin(beta + th1B + th2B + th3B) - 0.5000*L*a3B*dth3B*ml3B*sin(beta + th1B + th2B + th3B) - 0.5000*L*a1A*dalfa*ml1A*sin(beta + th1A) - L*a1A*dalfa*ml2A*sin(beta + th1A) - L*a1A*dalfa*ml3A*sin(beta + th1A) - 0.5000*L*a1B*dalfa*ml1B*sin(beta + th1B) - L*a1B*dalfa*ml2B*sin(beta + th1B) - L*a1B*dalfa*ml3B*sin(beta + th1B) - 0.5000*L*a1A*dbeta*ml1A*sin(beta + th1A) - L*a1A*dbeta*ml2A*sin(beta + th1A) - L*a1A*dbeta*ml3A*sin(beta + th1A) - 0.5000*L*a1B*dbeta*ml1B*sin(beta + th1B) - L*a1B*dbeta*ml2B*sin(beta + th1B) - L*a1B*dbeta*ml3B*sin(beta + th1B) - 0.5000*L*a1A*dth1A*ml1A*sin(beta + th1A) - L*a1A*dth1A*ml2A*sin(beta + th1A) - L*a1A*dth1A*ml3A*sin(beta + th1A) - 0.5000*L*a1B*dth1B*ml1B*sin(beta + th1B) - L*a1B*dth1B*ml2B*sin(beta + th1B) - L*a1B*dth1B*ml3B*sin(beta + th1B) - 0.5000*a1A*a3A*dth2A*ml3A*sin(th2A + th3A) - 0.5000*a1A*a3A*dth3A*ml3A*sin(th2A + th3A) - 0.5000*a1B*a3B*dth2B*ml3B*sin(th2B + th3B) - 0.5000*a1B*a3B*dth3B*ml3B*sin(th2B + th3B) - 0.5000*a2A*dth1A*ml2A*offA*sin(th1A + th2A) - a2A*dth1A*ml3A*offA*sin(th1A + th2A) - 0.5000*a2A*dth2A*ml2A*offA*sin(th1A + th2A) - a2A*dth2A*ml3A*offA*sin(th1A + th2A) - 0.5000*a2B*dth1B*ml2B*offB*sin(th1B + th2B) - a2B*dth1B*ml3B*offB*sin(th1B + th2B) - 0.5000*a2B*dth2B*ml2B*offB*sin(th1B + th2B) - a2B*dth2B*ml3B*offB*sin(th1B + th2B) - L*dalfa*ml1A*offA*sin(beta) - L*dalfa*ml2A*offA*sin(beta) - L*dalfa*ml1B*offB*sin(beta) - L*dalfa*ml3A*offA*sin(beta) - L*dalfa*ml2B*offB*sin(beta) - L*dalfa*ml3B*offB*sin(beta) - L*dbeta*ml1A*offA*sin(beta) - L*dbeta*ml2A*offA*sin(beta) - L*dbeta*ml1B*offB*sin(beta) - L*dbeta*ml3A*offA*sin(beta) - L*dbeta*ml2B*offB*sin(beta) - L*dbeta*ml3B*offB*sin(beta) - 0.5000*a1A*a2A*dth2A*ml2A*sin(th2A) - a1A*a2A*dth2A*ml3A*sin(th2A) - 0.5000*a2A*a3A*dth3A*ml3A*sin(th3A) - 0.5000*a1B*a2B*dth2B*ml2B*sin(th2B) - a1B*a2B*dth2B*ml3B*sin(th2B) - 0.5000*a2B*a3B*dth3B*ml3B*sin(th3B) - 0.5000*a1A*dth1A*ml1A*offA*sin(th1A) - a1A*dth1A*ml2A*offA*sin(th1A) - a1A*dth1A*ml3A*offA*sin(th1A) - 0.5000*a1B*dth1B*ml1B*offB*sin(th1B) - a1B*dth1B*ml2B*offB*sin(th1B) - a1B*dth1B*ml3B*offB*sin(th1B) - 0.5000*L*a2A*dalfa*ml2A*sin(beta + th1A + th2A) - L*a2A*dalfa*ml3A*sin(beta + th1A + th2A) - 0.5000*L*a2B*dalfa*ml2B*sin(beta + th1B + th2B) - L*a2B*dalfa*ml3B*sin(beta + th1B + th2B) - 0.5000*L*a2A*dbeta*ml2A*sin(beta + th1A + th2A) - L*a2A*dbeta*ml3A*sin(beta + th1A + th2A) - 0.5000*L*a2B*dbeta*ml2B*sin(beta + th1B + th2B) - L*a2B*dbeta*ml3B*sin(beta + th1B + th2B) - 0.5000*L*a2A*dth1A*ml2A*sin(beta + th1A + th2A) - L*a2A*dth1A*ml3A*sin(beta + th1A + th2A) - 0.5000*L*a2A*dth2A*ml2A*sin(beta + th1A + th2A) - L*a2A*dth2A*ml3A*sin(beta + th1A + th2A) - 0.5000*L*a2B*dth1B*ml2B*sin(beta + th1B + th2B) - L*a2B*dth1B*ml3B*sin(beta + th1B + th2B) - 0.5000*L*a2B*dth2B*ml2B*sin(beta + th1B + th2B) - L*a2B*dth2B*ml3B*sin(beta + th1B + th2B), - 0.5000*a3A*dalfa*ml3A*offA*sin(th1A + th2A + th3A) - 0.5000*a3A*dbeta*ml3A*offA*sin(th1A + th2A + th3A) - 0.5000*a3A*dth1A*ml3A*offA*sin(th1A + th2A + th3A) - 0.5000*a3A*dth2A*ml3A*offA*sin(th1A + th2A + th3A) - 0.5000*a3A*dth3A*ml3A*offA*sin(th1A + th2A + th3A) - 0.5000*L*a3A*dalfa*ml3A*sin(beta + th1A + th2A + th3A) - 0.5000*L*a3A*dbeta*ml3A*sin(beta + th1A + th2A + th3A) - 0.5000*L*a3A*dth1A*ml3A*sin(beta + th1A + th2A + th3A) - 0.5000*L*a3A*dth2A*ml3A*sin(beta + th1A + th2A + th3A) - 0.5000*L*a3A*dth3A*ml3A*sin(beta + th1A + th2A + th3A) - 0.5000*L*a1A*dalfa*ml1A*sin(beta + th1A) - L*a1A*dalfa*ml2A*sin(beta + th1A) - L*a1A*dalfa*ml3A*sin(beta + th1A) - 0.5000*L*a1A*dbeta*ml1A*sin(beta + th1A) - L*a1A*dbeta*ml2A*sin(beta + th1A) - L*a1A*dbeta*ml3A*sin(beta + th1A) - 0.5000*L*a1A*dth1A*ml1A*sin(beta + th1A) - L*a1A*dth1A*ml2A*sin(beta + th1A) - L*a1A*dth1A*ml3A*sin(beta + th1A) - 0.5000*a1A*a3A*dth2A*ml3A*sin(th2A + th3A) - 0.5000*a1A*a3A*dth3A*ml3A*sin(th2A + th3A) - 0.5000*a2A*dalfa*ml2A*offA*sin(th1A + th2A) - a2A*dalfa*ml3A*offA*sin(th1A + th2A) - 0.5000*a2A*dbeta*ml2A*offA*sin(th1A + th2A) - a2A*dbeta*ml3A*offA*sin(th1A + th2A) - 0.5000*a2A*dth1A*ml2A*offA*sin(th1A + th2A) - a2A*dth1A*ml3A*offA*sin(th1A + th2A) - 0.5000*a2A*dth2A*ml2A*offA*sin(th1A + th2A) - a2A*dth2A*ml3A*offA*sin(th1A + th2A) - 0.5000*a1A*a2A*dth2A*ml2A*sin(th2A) - a1A*a2A*dth2A*ml3A*sin(th2A) - 0.5000*a2A*a3A*dth3A*ml3A*sin(th3A) - 0.5000*a1A*dalfa*ml1A*offA*sin(th1A) - a1A*dalfa*ml2A*offA*sin(th1A) - a1A*dalfa*ml3A*offA*sin(th1A) - 0.5000*a1A*dbeta*ml1A*offA*sin(th1A) - a1A*dbeta*ml2A*offA*sin(th1A) - a1A*dbeta*ml3A*offA*sin(th1A) - 0.5000*a1A*dth1A*ml1A*offA*sin(th1A) - a1A*dth1A*ml2A*offA*sin(th1A) - a1A*dth1A*ml3A*offA*sin(th1A) - 0.5000*L*a2A*dalfa*ml2A*sin(beta + th1A + th2A) - L*a2A*dalfa*ml3A*sin(beta + th1A + th2A) - 0.5000*L*a2A*dbeta*ml2A*sin(beta + th1A + th2A) - L*a2A*dbeta*ml3A*sin(beta + th1A + th2A) - 0.5000*L*a2A*dth1A*ml2A*sin(beta + th1A + th2A) - L*a2A*dth1A*ml3A*sin(beta + th1A + th2A) - 0.5000*L*a2A*dth2A*ml2A*sin(beta + th1A + th2A) - L*a2A*dth2A*ml3A*sin(beta + th1A + th2A), - 0.5000*a3A*dalfa*ml3A*offA*sin(th1A + th2A + th3A) - 0.5000*a3A*dbeta*ml3A*offA*sin(th1A + th2A + th3A) - 0.5000*a3A*dth1A*ml3A*offA*sin(th1A + th2A + th3A) - 0.5000*a3A*dth2A*ml3A*offA*sin(th1A + th2A + th3A) - 0.5000*a3A*dth3A*ml3A*offA*sin(th1A + th2A + th3A) - 0.5000*L*a3A*dalfa*ml3A*sin(beta + th1A + th2A + th3A) - 0.5000*L*a3A*dbeta*ml3A*sin(beta + th1A + th2A + th3A) - 0.5000*L*a3A*dth1A*ml3A*sin(beta + th1A + th2A + th3A) - 0.5000*L*a3A*dth2A*ml3A*sin(beta + th1A + th2A + th3A) - 0.5000*L*a3A*dth3A*ml3A*sin(beta + th1A + th2A + th3A) - 0.5000*a1A*a3A*dalfa*ml3A*sin(th2A + th3A) - 0.5000*a1A*a3A*dbeta*ml3A*sin(th2A + th3A) - 0.5000*a1A*a3A*dth1A*ml3A*sin(th2A + th3A) - 0.5000*a1A*a3A*dth2A*ml3A*sin(th2A + th3A) - 0.5000*a1A*a3A*dth3A*ml3A*sin(th2A + th3A) - 0.5000*a2A*dalfa*ml2A*offA*sin(th1A + th2A) - a2A*dalfa*ml3A*offA*sin(th1A + th2A) - 0.5000*a2A*dbeta*ml2A*offA*sin(th1A + th2A) - a2A*dbeta*ml3A*offA*sin(th1A + th2A) - 0.5000*a2A*dth1A*ml2A*offA*sin(th1A + th2A) - a2A*dth1A*ml3A*offA*sin(th1A + th2A) - 0.5000*a2A*dth2A*ml2A*offA*sin(th1A + th2A) - a2A*dth2A*ml3A*offA*sin(th1A + th2A) - 0.5000*a1A*a2A*dalfa*ml2A*sin(th2A) - a1A*a2A*dalfa*ml3A*sin(th2A) - 0.5000*a1A*a2A*dbeta*ml2A*sin(th2A) - a1A*a2A*dbeta*ml3A*sin(th2A) - 0.5000*a1A*a2A*dth1A*ml2A*sin(th2A) - a1A*a2A*dth1A*ml3A*sin(th2A) - 0.5000*a1A*a2A*dth2A*ml2A*sin(th2A) - a1A*a2A*dth2A*ml3A*sin(th2A) - 0.5000*a2A*a3A*dth3A*ml3A*sin(th3A) - 0.5000*L*a2A*dalfa*ml2A*sin(beta + th1A + th2A) - L*a2A*dalfa*ml3A*sin(beta + th1A + th2A) - 0.5000*L*a2A*dbeta*ml2A*sin(beta + th1A + th2A) - L*a2A*dbeta*ml3A*sin(beta + th1A + th2A) - 0.5000*L*a2A*dth1A*ml2A*sin(beta + th1A + th2A) - L*a2A*dth1A*ml3A*sin(beta + th1A + th2A) - 0.5000*L*a2A*dth2A*ml2A*sin(beta + th1A + th2A) - L*a2A*dth2A*ml3A*sin(beta + th1A + th2A), -0.5000*a3A*ml3A*(L*sin(beta + th1A + th2A + th3A) + a1A*sin(th2A + th3A) + a2A*sin(th3A) + offA*sin(th1A + th2A + th3A))*(dalfa + dbeta + dth1A + dth2A + dth3A), - 0.5000*a3B*dalfa*ml3B*offB*sin(th1B + th2B + th3B) - 0.5000*a3B*dbeta*ml3B*offB*sin(th1B + th2B + th3B) - 0.5000*a3B*dth1B*ml3B*offB*sin(th1B + th2B + th3B) - 0.5000*a3B*dth2B*ml3B*offB*sin(th1B + th2B + th3B) - 0.5000*a3B*dth3B*ml3B*offB*sin(th1B + th2B + th3B) - 0.5000*L*a3B*dalfa*ml3B*sin(beta + th1B + th2B + th3B) - 0.5000*L*a3B*dbeta*ml3B*sin(beta + th1B + th2B + th3B) - 0.5000*L*a3B*dth1B*ml3B*sin(beta + th1B + th2B + th3B) - 0.5000*L*a3B*dth2B*ml3B*sin(beta + th1B + th2B + th3B) - 0.5000*L*a3B*dth3B*ml3B*sin(beta + th1B + th2B + th3B) - 0.5000*L*a1B*dalfa*ml1B*sin(beta + th1B) - L*a1B*dalfa*ml2B*sin(beta + th1B) - L*a1B*dalfa*ml3B*sin(beta + th1B) - 0.5000*L*a1B*dbeta*ml1B*sin(beta + th1B) - L*a1B*dbeta*ml2B*sin(beta + th1B) - L*a1B*dbeta*ml3B*sin(beta + th1B) - 0.5000*L*a1B*dth1B*ml1B*sin(beta + th1B) - L*a1B*dth1B*ml2B*sin(beta + th1B) - L*a1B*dth1B*ml3B*sin(beta + th1B) - 0.5000*a1B*a3B*dth2B*ml3B*sin(th2B + th3B) - 0.5000*a1B*a3B*dth3B*ml3B*sin(th2B + th3B) - 0.5000*a2B*dalfa*ml2B*offB*sin(th1B + th2B) - a2B*dalfa*ml3B*offB*sin(th1B + th2B) - 0.5000*a2B*dbeta*ml2B*offB*sin(th1B + th2B) - a2B*dbeta*ml3B*offB*sin(th1B + th2B) - 0.5000*a2B*dth1B*ml2B*offB*sin(th1B + th2B) - a2B*dth1B*ml3B*offB*sin(th1B + th2B) - 0.5000*a2B*dth2B*ml2B*offB*sin(th1B + th2B) - a2B*dth2B*ml3B*offB*sin(th1B + th2B) - 0.5000*a1B*a2B*dth2B*ml2B*sin(th2B) - a1B*a2B*dth2B*ml3B*sin(th2B) - 0.5000*a2B*a3B*dth3B*ml3B*sin(th3B) - 0.5000*a1B*dalfa*ml1B*offB*sin(th1B) - a1B*dalfa*ml2B*offB*sin(th1B) - a1B*dalfa*ml3B*offB*sin(th1B) - 0.5000*a1B*dbeta*ml1B*offB*sin(th1B) - a1B*dbeta*ml2B*offB*sin(th1B) - a1B*dbeta*ml3B*offB*sin(th1B) - 0.5000*a1B*dth1B*ml1B*offB*sin(th1B) - a1B*dth1B*ml2B*offB*sin(th1B) - a1B*dth1B*ml3B*offB*sin(th1B) - 0.5000*L*a2B*dalfa*ml2B*sin(beta + th1B + th2B) - L*a2B*dalfa*ml3B*sin(beta + th1B + th2B) - 0.5000*L*a2B*dbeta*ml2B*sin(beta + th1B + th2B) - L*a2B*dbeta*ml3B*sin(beta + th1B + th2B) - 0.5000*L*a2B*dth1B*ml2B*sin(beta + th1B + th2B) - L*a2B*dth1B*ml3B*sin(beta + th1B + th2B) - 0.5000*L*a2B*dth2B*ml2B*sin(beta + th1B + th2B) - L*a2B*dth2B*ml3B*sin(beta + th1B + th2B), - 0.5000*a3B*dalfa*ml3B*offB*sin(th1B + th2B + th3B) - 0.5000*a3B*dbeta*ml3B*offB*sin(th1B + th2B + th3B) - 0.5000*a3B*dth1B*ml3B*offB*sin(th1B + th2B + th3B) - 0.5000*a3B*dth2B*ml3B*offB*sin(th1B + th2B + th3B) - 0.5000*a3B*dth3B*ml3B*offB*sin(th1B + th2B + th3B) - 0.5000*L*a3B*dalfa*ml3B*sin(beta + th1B + th2B + th3B) - 0.5000*L*a3B*dbeta*ml3B*sin(beta + th1B + th2B + th3B) - 0.5000*L*a3B*dth1B*ml3B*sin(beta + th1B + th2B + th3B) - 0.5000*L*a3B*dth2B*ml3B*sin(beta + th1B + th2B + th3B) - 0.5000*L*a3B*dth3B*ml3B*sin(beta + th1B + th2B + th3B) - 0.5000*a1B*a3B*dalfa*ml3B*sin(th2B + th3B) - 0.5000*a1B*a3B*dbeta*ml3B*sin(th2B + th3B) - 0.5000*a1B*a3B*dth1B*ml3B*sin(th2B + th3B) - 0.5000*a1B*a3B*dth2B*ml3B*sin(th2B + th3B) - 0.5000*a1B*a3B*dth3B*ml3B*sin(th2B + th3B) - 0.5000*a2B*dalfa*ml2B*offB*sin(th1B + th2B) - a2B*dalfa*ml3B*offB*sin(th1B + th2B) - 0.5000*a2B*dbeta*ml2B*offB*sin(th1B + th2B) - a2B*dbeta*ml3B*offB*sin(th1B + th2B) - 0.5000*a2B*dth1B*ml2B*offB*sin(th1B + th2B) - a2B*dth1B*ml3B*offB*sin(th1B + th2B) - 0.5000*a2B*dth2B*ml2B*offB*sin(th1B + th2B) - a2B*dth2B*ml3B*offB*sin(th1B + th2B) - 0.5000*a1B*a2B*dalfa*ml2B*sin(th2B) - a1B*a2B*dalfa*ml3B*sin(th2B) - 0.5000*a1B*a2B*dbeta*ml2B*sin(th2B) - a1B*a2B*dbeta*ml3B*sin(th2B) - 0.5000*a1B*a2B*dth1B*ml2B*sin(th2B) - a1B*a2B*dth1B*ml3B*sin(th2B) - 0.5000*a1B*a2B*dth2B*ml2B*sin(th2B) - a1B*a2B*dth2B*ml3B*sin(th2B) - 0.5000*a2B*a3B*dth3B*ml3B*sin(th3B) - 0.5000*L*a2B*dalfa*ml2B*sin(beta + th1B + th2B) - L*a2B*dalfa*ml3B*sin(beta + th1B + th2B) - 0.5000*L*a2B*dbeta*ml2B*sin(beta + th1B + th2B) - L*a2B*dbeta*ml3B*sin(beta + th1B + th2B) - 0.5000*L*a2B*dth1B*ml2B*sin(beta + th1B + th2B) - L*a2B*dth1B*ml3B*sin(beta + th1B + th2B) - 0.5000*L*a2B*dth2B*ml2B*sin(beta + th1B + th2B) - L*a2B*dth2B*ml3B*sin(beta + th1B + th2B), -0.5000*a3B*ml3B*(L*sin(beta + th1B + th2B + th3B) + a1B*sin(th2B + th3B) + a2B*sin(th3B) + offB*sin(th1B + th2B + th3B))*(dalfa + dbeta + dth1B + dth2B + dth3B); ...
                                                                                                                                                                                                                                                                                                                                                                                                                                                                                                                                                                                                                                                                                                                                                                                                                                                                                                                                                                                        0.5000*L*a3A*dalfa*ml3A*sin(beta + th1A + th2A + th3A) - 0.5000*a3A*dth2A*ml3A*offA*sin(th1A + th2A + th3A) - 0.5000*a3A*dth3A*ml3A*offA*sin(th1A + th2A + th3A) - 0.5000*a3B*dth1B*ml3B*offB*sin(th1B + th2B + th3B) - 0.5000*a3B*dth2B*ml3B*offB*sin(th1B + th2B + th3B) - 0.5000*a3B*dth3B*ml3B*offB*sin(th1B + th2B + th3B) - 0.5000*a3A*dth1A*ml3A*offA*sin(th1A + th2A + th3A) + 0.5000*L*a3B*dalfa*ml3B*sin(beta + th1B + th2B + th3B) + 0.5000*L*a1A*dalfa*ml1A*sin(beta + th1A) + L*a1A*dalfa*ml2A*sin(beta + th1A) + L*a1A*dalfa*ml3A*sin(beta + th1A) + 0.5000*L*a1B*dalfa*ml1B*sin(beta + th1B) + L*a1B*dalfa*ml2B*sin(beta + th1B) + L*a1B*dalfa*ml3B*sin(beta + th1B) - 0.5000*a1A*a3A*dth2A*ml3A*sin(th2A + th3A) - 0.5000*a1A*a3A*dth3A*ml3A*sin(th2A + th3A) - 0.5000*a1B*a3B*dth2B*ml3B*sin(th2B + th3B) - 0.5000*a1B*a3B*dth3B*ml3B*sin(th2B + th3B) - 0.5000*a2A*dth1A*ml2A*offA*sin(th1A + th2A) - a2A*dth1A*ml3A*offA*sin(th1A + th2A) - 0.5000*a2A*dth2A*ml2A*offA*sin(th1A + th2A) - a2A*dth2A*ml3A*offA*sin(th1A + th2A) - 0.5000*a2B*dth1B*ml2B*offB*sin(th1B + th2B) - a2B*dth1B*ml3B*offB*sin(th1B + th2B) - 0.5000*a2B*dth2B*ml2B*offB*sin(th1B + th2B) - a2B*dth2B*ml3B*offB*sin(th1B + th2B) + L*dalfa*ml1A*offA*sin(beta) + L*dalfa*ml2A*offA*sin(beta) + L*dalfa*ml1B*offB*sin(beta) + L*dalfa*ml3A*offA*sin(beta) + L*dalfa*ml2B*offB*sin(beta) + L*dalfa*ml3B*offB*sin(beta) - 0.5000*a1A*a2A*dth2A*ml2A*sin(th2A) - a1A*a2A*dth2A*ml3A*sin(th2A) - 0.5000*a2A*a3A*dth3A*ml3A*sin(th3A) - 0.5000*a1B*a2B*dth2B*ml2B*sin(th2B) - a1B*a2B*dth2B*ml3B*sin(th2B) - 0.5000*a2B*a3B*dth3B*ml3B*sin(th3B) - 0.5000*a1A*dth1A*ml1A*offA*sin(th1A) - a1A*dth1A*ml2A*offA*sin(th1A) - a1A*dth1A*ml3A*offA*sin(th1A) - 0.5000*a1B*dth1B*ml1B*offB*sin(th1B) - a1B*dth1B*ml2B*offB*sin(th1B) - a1B*dth1B*ml3B*offB*sin(th1B) + 0.5000*L*a2A*dalfa*ml2A*sin(beta + th1A + th2A) + L*a2A*dalfa*ml3A*sin(beta + th1A + th2A) + 0.5000*L*a2B*dalfa*ml2B*sin(beta + th1B + th2B) + L*a2B*dalfa*ml3B*sin(beta + th1B + th2B),                                                                                                                                                                                                                                                                                                                                                                                                                                                                                                                                                                                                                                                                                                                                                                                                                                                                                                                                                                                                                                                                                                                                                                                                                                                                                                                                                                                                                                                                                                                                                                                                                                                                                                                                                                                                                                                                                                                                                                                                                                                                                                                                                                                                                                                                                                                                                                                                                                                             - 0.5000*a3A*dth1A*ml3A*offA*sin(th1A + th2A + th3A) - 0.5000*a3A*dth2A*ml3A*offA*sin(th1A + th2A + th3A) - 0.5000*a3A*dth3A*ml3A*offA*sin(th1A + th2A + th3A) - 0.5000*a3B*dth1B*ml3B*offB*sin(th1B + th2B + th3B) - 0.5000*a3B*dth2B*ml3B*offB*sin(th1B + th2B + th3B) - 0.5000*a3B*dth3B*ml3B*offB*sin(th1B + th2B + th3B) - 0.5000*a1A*a3A*dth2A*ml3A*sin(th2A + th3A) - 0.5000*a1A*a3A*dth3A*ml3A*sin(th2A + th3A) - 0.5000*a1B*a3B*dth2B*ml3B*sin(th2B + th3B) - 0.5000*a1B*a3B*dth3B*ml3B*sin(th2B + th3B) - 0.5000*a2A*dth1A*ml2A*offA*sin(th1A + th2A) - a2A*dth1A*ml3A*offA*sin(th1A + th2A) - 0.5000*a2A*dth2A*ml2A*offA*sin(th1A + th2A) - a2A*dth2A*ml3A*offA*sin(th1A + th2A) - 0.5000*a2B*dth1B*ml2B*offB*sin(th1B + th2B) - a2B*dth1B*ml3B*offB*sin(th1B + th2B) - 0.5000*a2B*dth2B*ml2B*offB*sin(th1B + th2B) - a2B*dth2B*ml3B*offB*sin(th1B + th2B) - 0.5000*a1A*a2A*dth2A*ml2A*sin(th2A) - a1A*a2A*dth2A*ml3A*sin(th2A) - 0.5000*a2A*a3A*dth3A*ml3A*sin(th3A) - 0.5000*a1B*a2B*dth2B*ml2B*sin(th2B) - a1B*a2B*dth2B*ml3B*sin(th2B) - 0.5000*a2B*a3B*dth3B*ml3B*sin(th3B) - 0.5000*a1A*dth1A*ml1A*offA*sin(th1A) - a1A*dth1A*ml2A*offA*sin(th1A) - a1A*dth1A*ml3A*offA*sin(th1A) - 0.5000*a1B*dth1B*ml1B*offB*sin(th1B) - a1B*dth1B*ml2B*offB*sin(th1B) - a1B*dth1B*ml3B*offB*sin(th1B),                                                                                                                                                                                                                                                                                                                                                                                                                                                                                                                                                                                                                                                                                                                                                                                                                                                                                                                                                                                                                                           - 0.5000*a3A*dalfa*ml3A*offA*sin(th1A + th2A + th3A) - 0.5000*a3A*dbeta*ml3A*offA*sin(th1A + th2A + th3A) - 0.5000*a3A*dth1A*ml3A*offA*sin(th1A + th2A + th3A) - 0.5000*a3A*dth2A*ml3A*offA*sin(th1A + th2A + th3A) - 0.5000*a3A*dth3A*ml3A*offA*sin(th1A + th2A + th3A) - 0.5000*a1A*a3A*dth2A*ml3A*sin(th2A + th3A) - 0.5000*a1A*a3A*dth3A*ml3A*sin(th2A + th3A) - 0.5000*a2A*dalfa*ml2A*offA*sin(th1A + th2A) - a2A*dalfa*ml3A*offA*sin(th1A + th2A) - 0.5000*a2A*dbeta*ml2A*offA*sin(th1A + th2A) - a2A*dbeta*ml3A*offA*sin(th1A + th2A) - 0.5000*a2A*dth1A*ml2A*offA*sin(th1A + th2A) - a2A*dth1A*ml3A*offA*sin(th1A + th2A) - 0.5000*a2A*dth2A*ml2A*offA*sin(th1A + th2A) - a2A*dth2A*ml3A*offA*sin(th1A + th2A) - 0.5000*a1A*a2A*dth2A*ml2A*sin(th2A) - a1A*a2A*dth2A*ml3A*sin(th2A) - 0.5000*a2A*a3A*dth3A*ml3A*sin(th3A) - 0.5000*a1A*dalfa*ml1A*offA*sin(th1A) - a1A*dalfa*ml2A*offA*sin(th1A) - a1A*dalfa*ml3A*offA*sin(th1A) - 0.5000*a1A*dbeta*ml1A*offA*sin(th1A) - a1A*dbeta*ml2A*offA*sin(th1A) - a1A*dbeta*ml3A*offA*sin(th1A) - 0.5000*a1A*dth1A*ml1A*offA*sin(th1A) - a1A*dth1A*ml2A*offA*sin(th1A) - a1A*dth1A*ml3A*offA*sin(th1A),                                                                                                                                                                                                                                                                                                                                                                                                                                                                                                                                                                                                                                                                                  - 0.5000*a3A*dalfa*ml3A*offA*sin(th1A + th2A + th3A) - 0.5000*a3A*dbeta*ml3A*offA*sin(th1A + th2A + th3A) - 0.5000*a3A*dth1A*ml3A*offA*sin(th1A + th2A + th3A) - 0.5000*a3A*dth2A*ml3A*offA*sin(th1A + th2A + th3A) - 0.5000*a3A*dth3A*ml3A*offA*sin(th1A + th2A + th3A) - 0.5000*a1A*a3A*dalfa*ml3A*sin(th2A + th3A) - 0.5000*a1A*a3A*dbeta*ml3A*sin(th2A + th3A) - 0.5000*a1A*a3A*dth1A*ml3A*sin(th2A + th3A) - 0.5000*a1A*a3A*dth2A*ml3A*sin(th2A + th3A) - 0.5000*a1A*a3A*dth3A*ml3A*sin(th2A + th3A) - 0.5000*a2A*dalfa*ml2A*offA*sin(th1A + th2A) - a2A*dalfa*ml3A*offA*sin(th1A + th2A) - 0.5000*a2A*dbeta*ml2A*offA*sin(th1A + th2A) - a2A*dbeta*ml3A*offA*sin(th1A + th2A) - 0.5000*a2A*dth1A*ml2A*offA*sin(th1A + th2A) - a2A*dth1A*ml3A*offA*sin(th1A + th2A) - 0.5000*a2A*dth2A*ml2A*offA*sin(th1A + th2A) - a2A*dth2A*ml3A*offA*sin(th1A + th2A) - 0.5000*a1A*a2A*dalfa*ml2A*sin(th2A) - a1A*a2A*dalfa*ml3A*sin(th2A) - 0.5000*a1A*a2A*dbeta*ml2A*sin(th2A) - a1A*a2A*dbeta*ml3A*sin(th2A) - 0.5000*a1A*a2A*dth1A*ml2A*sin(th2A) - a1A*a2A*dth1A*ml3A*sin(th2A) - 0.5000*a1A*a2A*dth2A*ml2A*sin(th2A) - a1A*a2A*dth2A*ml3A*sin(th2A) - 0.5000*a2A*a3A*dth3A*ml3A*sin(th3A),                                    -0.5000*a3A*ml3A*(a1A*sin(th2A + th3A) + a2A*sin(th3A) + offA*sin(th1A + th2A + th3A))*(dalfa + dbeta + dth1A + dth2A + dth3A),                                                                                                                                                                                                                                                                                                                                                                                                                                                                                                                                                                                                                                                                                                                                                                                                                                                                                                                                                                                                                                           - 0.5000*a3B*dalfa*ml3B*offB*sin(th1B + th2B + th3B) - 0.5000*a3B*dbeta*ml3B*offB*sin(th1B + th2B + th3B) - 0.5000*a3B*dth1B*ml3B*offB*sin(th1B + th2B + th3B) - 0.5000*a3B*dth2B*ml3B*offB*sin(th1B + th2B + th3B) - 0.5000*a3B*dth3B*ml3B*offB*sin(th1B + th2B + th3B) - 0.5000*a1B*a3B*dth2B*ml3B*sin(th2B + th3B) - 0.5000*a1B*a3B*dth3B*ml3B*sin(th2B + th3B) - 0.5000*a2B*dalfa*ml2B*offB*sin(th1B + th2B) - a2B*dalfa*ml3B*offB*sin(th1B + th2B) - 0.5000*a2B*dbeta*ml2B*offB*sin(th1B + th2B) - a2B*dbeta*ml3B*offB*sin(th1B + th2B) - 0.5000*a2B*dth1B*ml2B*offB*sin(th1B + th2B) - a2B*dth1B*ml3B*offB*sin(th1B + th2B) - 0.5000*a2B*dth2B*ml2B*offB*sin(th1B + th2B) - a2B*dth2B*ml3B*offB*sin(th1B + th2B) - 0.5000*a1B*a2B*dth2B*ml2B*sin(th2B) - a1B*a2B*dth2B*ml3B*sin(th2B) - 0.5000*a2B*a3B*dth3B*ml3B*sin(th3B) - 0.5000*a1B*dalfa*ml1B*offB*sin(th1B) - a1B*dalfa*ml2B*offB*sin(th1B) - a1B*dalfa*ml3B*offB*sin(th1B) - 0.5000*a1B*dbeta*ml1B*offB*sin(th1B) - a1B*dbeta*ml2B*offB*sin(th1B) - a1B*dbeta*ml3B*offB*sin(th1B) - 0.5000*a1B*dth1B*ml1B*offB*sin(th1B) - a1B*dth1B*ml2B*offB*sin(th1B) - a1B*dth1B*ml3B*offB*sin(th1B),                                                                                                                                                                                                                                                                                                                                                                                                                                                                                                                                                                                                                                                                                  - 0.5000*a3B*dalfa*ml3B*offB*sin(th1B + th2B + th3B) - 0.5000*a3B*dbeta*ml3B*offB*sin(th1B + th2B + th3B) - 0.5000*a3B*dth1B*ml3B*offB*sin(th1B + th2B + th3B) - 0.5000*a3B*dth2B*ml3B*offB*sin(th1B + th2B + th3B) - 0.5000*a3B*dth3B*ml3B*offB*sin(th1B + th2B + th3B) - 0.5000*a1B*a3B*dalfa*ml3B*sin(th2B + th3B) - 0.5000*a1B*a3B*dbeta*ml3B*sin(th2B + th3B) - 0.5000*a1B*a3B*dth1B*ml3B*sin(th2B + th3B) - 0.5000*a1B*a3B*dth2B*ml3B*sin(th2B + th3B) - 0.5000*a1B*a3B*dth3B*ml3B*sin(th2B + th3B) - 0.5000*a2B*dalfa*ml2B*offB*sin(th1B + th2B) - a2B*dalfa*ml3B*offB*sin(th1B + th2B) - 0.5000*a2B*dbeta*ml2B*offB*sin(th1B + th2B) - a2B*dbeta*ml3B*offB*sin(th1B + th2B) - 0.5000*a2B*dth1B*ml2B*offB*sin(th1B + th2B) - a2B*dth1B*ml3B*offB*sin(th1B + th2B) - 0.5000*a2B*dth2B*ml2B*offB*sin(th1B + th2B) - a2B*dth2B*ml3B*offB*sin(th1B + th2B) - 0.5000*a1B*a2B*dalfa*ml2B*sin(th2B) - a1B*a2B*dalfa*ml3B*sin(th2B) - 0.5000*a1B*a2B*dbeta*ml2B*sin(th2B) - a1B*a2B*dbeta*ml3B*sin(th2B) - 0.5000*a1B*a2B*dth1B*ml2B*sin(th2B) - a1B*a2B*dth1B*ml3B*sin(th2B) - 0.5000*a1B*a2B*dth2B*ml2B*sin(th2B) - a1B*a2B*dth2B*ml3B*sin(th2B) - 0.5000*a2B*a3B*dth3B*ml3B*sin(th3B),                                    -0.5000*a3B*ml3B*(a1B*sin(th2B + th3B) + a2B*sin(th3B) + offB*sin(th1B + th2B + th3B))*(dalfa + dbeta + dth1B + dth2B + dth3B); ...
                                                                                                                                                                                                                                                                                                                                                                                                                                                                                                                                                                                                                                                                                                                                                                                                                                                                                                                                                                                                                                                                                                                                                                                                                                                                                                                                                                                                                                                                                                                                                                                                                                                                                                                                                                                                                                                                                                                                                                                                                                                        0.5000*a3A*dalfa*ml3A*offA*sin(th1A + th2A + th3A) + 0.5000*a3A*dbeta*ml3A*offA*sin(th1A + th2A + th3A) + 0.5000*L*a3A*dalfa*ml3A*sin(beta + th1A + th2A + th3A) + 0.5000*L*a1A*dalfa*ml1A*sin(beta + th1A) + L*a1A*dalfa*ml2A*sin(beta + th1A) + L*a1A*dalfa*ml3A*sin(beta + th1A) - 0.5000*a1A*a3A*dth2A*ml3A*sin(th2A + th3A) - 0.5000*a1A*a3A*dth3A*ml3A*sin(th2A + th3A) + 0.5000*a2A*dalfa*ml2A*offA*sin(th1A + th2A) + a2A*dalfa*ml3A*offA*sin(th1A + th2A) + 0.5000*a2A*dbeta*ml2A*offA*sin(th1A + th2A) + a2A*dbeta*ml3A*offA*sin(th1A + th2A) - 0.5000*a1A*a2A*dth2A*ml2A*sin(th2A) - a1A*a2A*dth2A*ml3A*sin(th2A) - 0.5000*a2A*a3A*dth3A*ml3A*sin(th3A) + 0.5000*a1A*dalfa*ml1A*offA*sin(th1A) + a1A*dalfa*ml2A*offA*sin(th1A) + a1A*dalfa*ml3A*offA*sin(th1A) + 0.5000*a1A*dbeta*ml1A*offA*sin(th1A) + a1A*dbeta*ml2A*offA*sin(th1A) + a1A*dbeta*ml3A*offA*sin(th1A) + 0.5000*L*a2A*dalfa*ml2A*sin(beta + th1A + th2A) + L*a2A*dalfa*ml3A*sin(beta + th1A + th2A),                                                                                                                                                                                                                                                                                                                                                                                                                                                                                                                                                                                                                                                                                                                                                                                                                                                                                                                                                                                                                                                                                                                                                                                                                                                                                                                                                                                                                                                                                                                                                                                                                                                                                                                                                                                                                                                                                                                                                                                                                                                                                                                                                                                                                                                                                                                                                                                                                                                                                                                                                                                                                                                                                                                                                                                                                                                                                                                                                                                                                                                                                                                                        dalfa*(0.5000*a2A*ml2A*offA*sin(th1A + th2A) + a2A*ml3A*offA*sin(th1A + th2A) + 0.5000*a1A*ml1A*offA*sin(th1A) + a1A*ml2A*offA*sin(th1A) + a1A*ml3A*offA*sin(th1A) + 0.5000*a3A*ml3A*offA*sin(th1A + th2A + th3A)) - dth2A*(0.5000*a1A*a3A*ml3A*sin(th2A + th3A) + 0.5000*a1A*a2A*ml2A*sin(th2A) + a1A*a2A*ml3A*sin(th2A)) - dth3A*(0.5000*a1A*a3A*ml3A*sin(th2A + th3A) + 0.5000*a2A*a3A*ml3A*sin(th3A)) + dbeta*(0.5000*a2A*ml2A*offA*sin(th1A + th2A) + a2A*ml3A*offA*sin(th1A + th2A) + 0.5000*a1A*ml1A*offA*sin(th1A) + a1A*ml2A*offA*sin(th1A) + a1A*ml3A*offA*sin(th1A) + 0.5000*a3A*ml3A*offA*sin(th1A + th2A + th3A)),                                                                                                                                                                                                                                                                                                                                                                                                                                                                                                                                                                                                                                                                                                                                                                                                                                                                                                                                                                                                                                                                                                                                                                                                                                                                                                                                                                                                                                                                                                                                                                                                                                                                                                                                                                                                                                                                                                                                                                                                           - dth3A*(0.5000*a1A*a3A*ml3A*sin(th2A + th3A) + 0.5000*a2A*a3A*ml3A*sin(th3A)) - dth2A*(0.5000*a1A*a3A*ml3A*sin(th2A + th3A) + 0.5000*a1A*a2A*ml2A*sin(th2A) + a1A*a2A*ml3A*sin(th2A)),                                                                                                                                                                                                                                                                                                                                                                                                                                                                                                                                                                                                                                                                                                                                                                                                                                                                                                                                                                                                                                                                                                                                                                                                                                                                                                                                                                                                                               - 0.5000*a1A*dalfa*(a2A*ml2A*sin(th2A) + 2*a2A*ml3A*sin(th2A) + a3A*ml3A*sin(th2A + th3A)) - 0.5000*a1A*dbeta*(a2A*ml2A*sin(th2A) + 2*a2A*ml3A*sin(th2A) + a3A*ml3A*sin(th2A + th3A)) - 0.5000*a1A*dth1A*(a2A*ml2A*sin(th2A) + 2*a2A*ml3A*sin(th2A) + a3A*ml3A*sin(th2A + th3A)) - 0.5000*a1A*dth2A*(a2A*ml2A*sin(th2A) + 2*a2A*ml3A*sin(th2A) + a3A*ml3A*sin(th2A + th3A)) - 0.5000*a3A*dth3A*ml3A*(a1A*sin(th2A + th3A) + a2A*sin(th3A)),                                                                   -0.5000*a3A*ml3A*(a1A*sin(th2A + th3A) + a2A*sin(th3A))*(dalfa + dbeta + dth1A + dth2A + dth3A),                                                                                                                                                                                                                                                                                                                                                                                                                                                                                                                                                                                                                                                                                                                                                                                                                                                                                                                                                                                                                                                                                                                                                                                                                                                                                                                                                                                                                                                                                                                                                                                                                                                                                                                                                                                                                                                                                                                                                                                                                                                                                                                                                                                                0,                                                                                                                                                                                                                                                                                                                                                                                                                                                                                                                                                                                                                                                                                                                                                                                                                                                                                                                                                                                                                                                                                                                                                                                                                                                                                                                                                                                                                                                                                                                                                                                                                                                                                                                                                                                                                                                                        0,                                                                                                                                                                 0; ...
                                                                                                                                                                                                                                                                                                                                                                                                                                                                                                                                                                                                                                                                                                                                                                                                                                                                                                                                                                                                                                                                                                                                                                                                                                                                                                                                                                                                                                                                                                                                                                                                                                                                                                                                                                                                                                                                                                                                                                                                                                                                                                                                                                                                  0.5000*a3A*dalfa*ml3A*offA*sin(th1A + th2A + th3A) + 0.5000*a3A*dbeta*ml3A*offA*sin(th1A + th2A + th3A) + 0.5000*L*a3A*dalfa*ml3A*sin(beta + th1A + th2A + th3A) + 0.5000*a1A*a3A*dalfa*ml3A*sin(th2A + th3A) + 0.5000*a1A*a3A*dbeta*ml3A*sin(th2A + th3A) + 0.5000*a1A*a3A*dth1A*ml3A*sin(th2A + th3A) + 0.5000*a2A*dalfa*ml2A*offA*sin(th1A + th2A) + a2A*dalfa*ml3A*offA*sin(th1A + th2A) + 0.5000*a2A*dbeta*ml2A*offA*sin(th1A + th2A) + a2A*dbeta*ml3A*offA*sin(th1A + th2A) + 0.5000*a1A*a2A*dalfa*ml2A*sin(th2A) + a1A*a2A*dalfa*ml3A*sin(th2A) + 0.5000*a1A*a2A*dbeta*ml2A*sin(th2A) + a1A*a2A*dbeta*ml3A*sin(th2A) + 0.5000*a1A*a2A*dth1A*ml2A*sin(th2A) + a1A*a2A*dth1A*ml3A*sin(th2A) - 0.5000*a2A*a3A*dth3A*ml3A*sin(th3A) + 0.5000*L*a2A*dalfa*ml2A*sin(beta + th1A + th2A) + L*a2A*dalfa*ml3A*sin(beta + th1A + th2A),                                                                                                                                                                                                                                                                                                                                                                                                                                                                                                                                                                                                                                                                                                                                                                                                                                                                                                                                                                                                                                                                                                                                                                                                                                                                                                                                                                                                                                                                                                                                                                                                                                                                                                                                                                                                                                                                                                                                                                                                                                                                                                                                                                                                                                                                                                                                                                                                                                                                                                                                                                                                                                                                                                                                                                                                                                                                                                                                                                                                                                                                                         0.5000*a3A*dalfa*ml3A*offA*sin(th1A + th2A + th3A) + 0.5000*a3A*dbeta*ml3A*offA*sin(th1A + th2A + th3A) + 0.5000*a1A*a3A*dalfa*ml3A*sin(th2A + th3A) + 0.5000*a1A*a3A*dbeta*ml3A*sin(th2A + th3A) + 0.5000*a1A*a3A*dth1A*ml3A*sin(th2A + th3A) + 0.5000*a2A*dalfa*ml2A*offA*sin(th1A + th2A) + a2A*dalfa*ml3A*offA*sin(th1A + th2A) + 0.5000*a2A*dbeta*ml2A*offA*sin(th1A + th2A) + a2A*dbeta*ml3A*offA*sin(th1A + th2A) + 0.5000*a1A*a2A*dalfa*ml2A*sin(th2A) + a1A*a2A*dalfa*ml3A*sin(th2A) + 0.5000*a1A*a2A*dbeta*ml2A*sin(th2A) + a1A*a2A*dbeta*ml3A*sin(th2A) + 0.5000*a1A*a2A*dth1A*ml2A*sin(th2A) + a1A*a2A*dth1A*ml3A*sin(th2A) - 0.5000*a2A*a3A*dth3A*ml3A*sin(th3A),                                                                                                                                                                                                                                                                                                                                                                                                                                                                                                                                                                                                                                                                                                                                                                                                                                                                                                                                                                                                                                                                                                                                                                                                                                                                                                                                                                                                                                                                                                                                                                                                                                                                                                                                                                                                                                                                             0.5000*a1A*dalfa*(a2A*ml2A*sin(th2A) + 2*a2A*ml3A*sin(th2A) + a3A*ml3A*sin(th2A + th3A)) + 0.5000*a1A*dbeta*(a2A*ml2A*sin(th2A) + 2*a2A*ml3A*sin(th2A) + a3A*ml3A*sin(th2A + th3A)) + 0.5000*a1A*dth1A*(a2A*ml2A*sin(th2A) + 2*a2A*ml3A*sin(th2A) + a3A*ml3A*sin(th2A + th3A)) - 0.5000*a2A*a3A*dth3A*ml3A*sin(th3A),                                                                                                                                                                                                                                                                                                                                                                                                                                                                                                                                                                                                                                                                                                                                                                                                                                                                                                                                                                                                                                                                                                                                                                                                                                                                                                                                                                                                                                                                                                                                                                                                                                                                                                                                                                                                                                     -0.5000*a2A*a3A*dth3A*ml3A*sin(th3A),                                                                                            -0.5000*a2A*a3A*ml3A*sin(th3A)*(dalfa + dbeta + dth1A + dth2A + dth3A),                                                                                                                                                                                                                                                                                                                                                                                                                                                                                                                                                                                                                                                                                                                                                                                                                                                                                                                                                                                                                                                                                                                                                                                                                                                                                                                                                                                                                                                                                                                                                                                                                                                                                                                                                                                                                                                                                                                                                                                                                                                                                                                                                                                                0,                                                                                                                                                                                                                                                                                                                                                                                                                                                                                                                                                                                                                                                                                                                                                                                                                                                                                                                                                                                                                                                                                                                                                                                                                                                                                                                                                                                                                                                                                                                                                                                                                                                                                                                                                                                                                                                                        0,                                                                                                                                                                 0; ...
                                                                                                                                                                                                                                                                                                                                                                                                                                                                                                                                                                                                                                                                                                                                                                                                                                                                                                                                                                                                                                                                                                                                                                                                                                                                                                                                                                                                                                                                                                                                                                                                                                                                                                                                                                                                                                                                                                                                                                                                                                                                                                                                                                                                                                                                                                                                                                                                                                                                                                                                                                                                                                                                                                                    0.5000*a3A*ml3A*(a2A*dalfa*sin(th3A) + a2A*dbeta*sin(th3A) + a2A*dth1A*sin(th3A) + a2A*dth2A*sin(th3A) + dalfa*offA*sin(th1A + th2A + th3A) + dbeta*offA*sin(th1A + th2A + th3A) + L*dalfa*sin(beta + th1A + th2A + th3A) + a1A*dalfa*sin(th2A + th3A) + a1A*dbeta*sin(th2A + th3A) + a1A*dth1A*sin(th2A + th3A)),                                                                                                                                                                                                                                                                                                                                                                                                                                                                                                                                                                                                                                                                                                                                                                                                                                                                                                                                                                                                                                                                                                                                                                                                                                                                                                                                                                                                                                                                                                                                                                                                                                                                                                                                                                                                                                                                                                                                                                                                                                                                                                                                                                                                                                                                                                                                                                                                                                                                                                                                                                                                                                                                                                                                                                                                                                                                                                                                                                                                                                                                                                                                                                                                                                                                                                                                                                                                                                                                                              0.5000*a3A*ml3A*(a2A*dalfa*sin(th3A) + a2A*dbeta*sin(th3A) + a2A*dth1A*sin(th3A) + a2A*dth2A*sin(th3A) + dalfa*offA*sin(th1A + th2A + th3A) + dbeta*offA*sin(th1A + th2A + th3A) + a1A*dalfa*sin(th2A + th3A) + a1A*dbeta*sin(th2A + th3A) + a1A*dth1A*sin(th2A + th3A)),                                                                                                                                                                                                                                                                                                                                                                                                                                                                                                                                                                                                                                                                                                                                                                                                                                                                                                                                                                                                                                                                                                                                                                                                                                                                                                                                                                                                                                                                                                                                                                                                                                                                                                                                                                                                                                                                                                                                                                                                   0.5000*a3A*ml3A*(a2A*dalfa*sin(th3A) + a2A*dbeta*sin(th3A) + a2A*dth1A*sin(th3A) + a2A*dth2A*sin(th3A) + a1A*dalfa*sin(th2A + th3A) + a1A*dbeta*sin(th2A + th3A) + a1A*dth1A*sin(th2A + th3A)),                                                                                                                                                                                                                                                                                                                                                                                                                                                                                                                                                                                                                                                                                                                                                                                                                                                                                                                                                                                                                                                                                                                                                                                                                                                                                                                                                                                                                                                                                                                                                                                                                                                                                                                                                                                                            0.5000*a2A*a3A*ml3A*sin(th3A)*(dalfa + dbeta + dth1A + dth2A),                                                                                                                                                                 0,                                                                                                                                                                                                                                                                                                                                                                                                                                                                                                                                                                                                                                                                                                                                                                                                                                                                                                                                                                                                                                                                                                                                                                                                                                                                                                                                                                                                                                                                                                                                                                                                                                                                                                                                                                                                                                                                                                                                                                                                                                                                                                                                                                                                0,                                                                                                                                                                                                                                                                                                                                                                                                                                                                                                                                                                                                                                                                                                                                                                                                                                                                                                                                                                                                                                                                                                                                                                                                                                                                                                                                                                                                                                                                                                                                                                                                                                                                                                                                                                                                                                                                        0,                                                                                                                                                                 0; ...
                                                                                                                                                                                                                                                                                                                                                                                                                                                                                                                                                                                                                                                                                                                                                                                                                                                                                                                                                                                                                                                                                                                                                                                                                                                                                                                                                                                                                                                                                                                                                                                                                                                                                                                                                                                                                                                                                                                                                                                                                                                        0.5000*a3B*dalfa*ml3B*offB*sin(th1B + th2B + th3B) + 0.5000*a3B*dbeta*ml3B*offB*sin(th1B + th2B + th3B) + 0.5000*L*a3B*dalfa*ml3B*sin(beta + th1B + th2B + th3B) + 0.5000*L*a1B*dalfa*ml1B*sin(beta + th1B) + L*a1B*dalfa*ml2B*sin(beta + th1B) + L*a1B*dalfa*ml3B*sin(beta + th1B) - 0.5000*a1B*a3B*dth2B*ml3B*sin(th2B + th3B) - 0.5000*a1B*a3B*dth3B*ml3B*sin(th2B + th3B) + 0.5000*a2B*dalfa*ml2B*offB*sin(th1B + th2B) + a2B*dalfa*ml3B*offB*sin(th1B + th2B) + 0.5000*a2B*dbeta*ml2B*offB*sin(th1B + th2B) + a2B*dbeta*ml3B*offB*sin(th1B + th2B) - 0.5000*a1B*a2B*dth2B*ml2B*sin(th2B) - a1B*a2B*dth2B*ml3B*sin(th2B) - 0.5000*a2B*a3B*dth3B*ml3B*sin(th3B) + 0.5000*a1B*dalfa*ml1B*offB*sin(th1B) + a1B*dalfa*ml2B*offB*sin(th1B) + a1B*dalfa*ml3B*offB*sin(th1B) + 0.5000*a1B*dbeta*ml1B*offB*sin(th1B) + a1B*dbeta*ml2B*offB*sin(th1B) + a1B*dbeta*ml3B*offB*sin(th1B) + 0.5000*L*a2B*dalfa*ml2B*sin(beta + th1B + th2B) + L*a2B*dalfa*ml3B*sin(beta + th1B + th2B),                                                                                                                                                                                                                                                                                                                                                                                                                                                                                                                                                                                                                                                                                                                                                                                                                                                                                                                                                                                                                                                                                                                                                                                                                                                                                                                                                                                                                                                                                                                                                                                                                                                                                                                                                                                                                                                                                                                                                                                                                                                                                                                                                                                                                                                                                                                                                                                                                                                                                                                                                                                                                                                                                                                                                                                                                                                                                                                                                                                                                                                                                                                                        dalfa*(0.5000*a2B*ml2B*offB*sin(th1B + th2B) + a2B*ml3B*offB*sin(th1B + th2B) + 0.5000*a1B*ml1B*offB*sin(th1B) + a1B*ml2B*offB*sin(th1B) + a1B*ml3B*offB*sin(th1B) + 0.5000*a3B*ml3B*offB*sin(th1B + th2B + th3B)) - dth2B*(0.5000*a1B*a3B*ml3B*sin(th2B + th3B) + 0.5000*a1B*a2B*ml2B*sin(th2B) + a1B*a2B*ml3B*sin(th2B)) - dth3B*(0.5000*a1B*a3B*ml3B*sin(th2B + th3B) + 0.5000*a2B*a3B*ml3B*sin(th3B)) + dbeta*(0.5000*a2B*ml2B*offB*sin(th1B + th2B) + a2B*ml3B*offB*sin(th1B + th2B) + 0.5000*a1B*ml1B*offB*sin(th1B) + a1B*ml2B*offB*sin(th1B) + a1B*ml3B*offB*sin(th1B) + 0.5000*a3B*ml3B*offB*sin(th1B + th2B + th3B)),                                                                                                                                                                                                                                                                                                                                                                                                                                                                                                                                                                                                                                                                                                                                                                                                                                                                                                                                                                                                                                                                                                                                                                                                                                                                                                                                                                                                                                                                                                                                                                                                                                                                                                                                                                                                                                                                                                                                                                                                                                                                                                                                                                                                0,                                                                                                                                                                                                                                                                                                                                                                                                                                                                                                                                                                                                                                                                                                                                                                                                                                                                                                                                                                                                                                                                                                                                                                                                                                                                                                                                                                                                                                                                                                                                                                                                                                                                                                                                                                                                                                                                        0,                                                                                                                                                                 0,                                                                                                                                                                                                                                                                                                                                                                                                                                                                                                                                                                                                                                                                                                                                                                                                                                                                                                                                                                                                                                                                                                                                                                                                                                                                                                                                                                                                                                                                                                                                                                                                                                                                                                                                                                                                                                                                                                                                                                                                           - dth3B*(0.5000*a1B*a3B*ml3B*sin(th2B + th3B) + 0.5000*a2B*a3B*ml3B*sin(th3B)) - dth2B*(0.5000*a1B*a3B*ml3B*sin(th2B + th3B) + 0.5000*a1B*a2B*ml2B*sin(th2B) + a1B*a2B*ml3B*sin(th2B)),                                                                                                                                                                                                                                                                                                                                                                                                                                                                                                                                                                                                                                                                                                                                                                                                                                                                                                                                                                                                                                                                                                                                                                                                                                                                                                                                                                                                                               - 0.5000*a1B*dalfa*(a2B*ml2B*sin(th2B) + 2*a2B*ml3B*sin(th2B) + a3B*ml3B*sin(th2B + th3B)) - 0.5000*a1B*dbeta*(a2B*ml2B*sin(th2B) + 2*a2B*ml3B*sin(th2B) + a3B*ml3B*sin(th2B + th3B)) - 0.5000*a1B*dth1B*(a2B*ml2B*sin(th2B) + 2*a2B*ml3B*sin(th2B) + a3B*ml3B*sin(th2B + th3B)) - 0.5000*a1B*dth2B*(a2B*ml2B*sin(th2B) + 2*a2B*ml3B*sin(th2B) + a3B*ml3B*sin(th2B + th3B)) - 0.5000*a3B*dth3B*ml3B*(a1B*sin(th2B + th3B) + a2B*sin(th3B)),                                                                   -0.5000*a3B*ml3B*(a1B*sin(th2B + th3B) + a2B*sin(th3B))*(dalfa + dbeta + dth1B + dth2B + dth3B); ...
